simulink model "pulsar_channeliser"  (R2012b)
(part 2 of 105)

      mask prompts: vec_len "Vector length:"; arith_type "Output type:"; n_bits "Bit width (output):"; bin_pt "Binary point (output):"
      mask help: This simple vector accumulator is based on a shift register. It outputs its previous accumulated vector after a new_acc pulse is received.
      mask init:
      | simple_bram_vacc_init(gcb, ...
      |     'vec_len', vec_len, ...
      |     'arith_type', arith_type, ...
      |     'n_bits', n_bits, ...
      |     'bin_pt', bin_pt);
      mask TypeOptions arith_type: Signed | Unsigned
  simple_bram_vacc_q_odd : Subsystem  AncestorBlock=casper_library_accumulators/simple_bram_vacc  mask(simple_bram_vacc){vec_len=32, arith_type=Signed, n_bits=32, bin_pt=17}
      mask prompts: vec_len "Vector length:"; arith_type "Output type:"; n_bits "Bit width (output):"; bin_pt "Binary point (output):"
      mask help: This simple vector accumulator is based on a shift register. It outputs its previous accumulated vector after a new_acc pulse is received.
      mask init:
      | simple_bram_vacc_init(gcb, ...
      |     'vec_len', vec_len, ...
      |     'arith_type', arith_type, ...
      |     'n_bits', n_bits, ...
      |     'bin_pt', bin_pt);
      mask TypeOptions arith_type: Signed | Unsigned
  spead_pack_btm : Subsystem  Tag=casper:spead_pack  AncestorBlock=casper_library_communications/spead_pack  mask(pkt_pack_mask){max_pkt_len_bits=10, header_ids=0x1601, 0x1700, header_ind_ids=0x1800, spead_msw=64, spead_lsw=40, spead_version=4, bytes_per_word=8}
      mask prompts: max_pkt_len_bits "Max pkt length, 2^? 64-bit words"; header_ids "SPEAD direct address IDs (decimal)"; header_ind_ids "SPEAD indirect address IDs (decimal)"; spead_msw "SPEAD Flavour (MSw)"; spead_lsw "SPEAD Flavour (LSw)"; spead_version "SPEAD version"; bytes_per_word "Word size, in bytes"
      mask help:
      | This block generates SPEAD-compliant packets from a datastream.
      |
      | Packets are created with a fixed header followed by a number of 64-bit items.
      |
      | Requires a 64-bit data stream.
      |
      | The data_ready signal is one cycle BEFORE valid data! Does not have to be with a valid signal either.
      mask init:
      | if floor(log2(bytes_per_word)) ~= log2(bytes_per_word)
      |     error('Bytes per word should be a power of two.');
      | end
      | 
      | spead_pack_init(gcb)
  spead_pack_top : Subsystem  Tag=casper:spead_pack  AncestorBlock=casper_library_communications/spead_pack  mask(pkt_pack_mask){max_pkt_len_bits=10, header_ids=0x1601, 0x1700, header_ind_ids=0x1800, spead_msw=64, spead_lsw=40, spead_version=4, bytes_per_word=8}
      mask prompts: max_pkt_len_bits "Max pkt length, 2^? 64-bit words"; header_ids "SPEAD direct address IDs (decimal)"; header_ind_ids "SPEAD indirect address IDs (decimal)"; spead_msw "SPEAD Flavour (MSw)"; spead_lsw "SPEAD Flavour (LSw)"; spead_version "SPEAD version"; bytes_per_word "Word size, in bytes"
      mask help:
      | This block generates SPEAD-compliant packets from a datastream.
      |
      | Packets are created with a fixed header followed by a number of 64-bit items.
      |
      | Requires a 64-bit data stream.
      |
      | The data_ready signal is one cycle BEFORE valid data! Does not have to be with a valid signal either.
      mask init:
      | if floor(log2(bytes_per_word)) ~= log2(bytes_per_word)
      |     error('Bytes per word should be a power of two.');
      | end
      | 
      | spead_pack_init(gcb)
  status_reg_ctrl : Subsystem  Tag=xps:sw_reg  AncestorBlock=xps_library/software register  DataTypeOverride=Double  DataTypeOverrideAppliesTo=Fixed-point  MinMaxOverflowLogging=ForceOff  mask(swreg){mode=one value, io_dir=From Processor, io_delay=0, sample_period=1, names=of_reset, bitwidths=1, arith_types=2, bin_pts=0, sim_port=on, show_format=off}
      mask prompts: io_dir "I/O direction"; io_delay "I/O delay"; sample_period "Sample period"; names "Name:"; bitwidths "Bitwidth:"; arith_types "Type (ufix=0, fix=1, bool=2):"; bin_pts "Binary pt:"; sim_port "Provide sim input/output?"; show_format "Print format string?"
      mask init:
      | swreg_init(gcb)
      settings: AttributesFormatString=1input
      mask TypeOptions mode: one value | fields of equal size | fields of arbitrary size
      mask Callback mode: swreg_cb(gcb);
      mask TypeOptions io_dir: To Processor | From Processor
      mask Callback io_dir:
      | mask_enables = get_param(gcb, 'MaskEnables');
      | mask_names = get_param(gcb, 'MaskNames');
      | if strcmp(get_param(gcb, 'io_dir'), 'To Processor'),
      |     mask_enables{ismember(mask_names, 'sample_period')} = 'off';
      | else
      |     mask_enables{ismember(mask_names, 'sample_period')} = 'on';
      | end
      | set_param(gcb, 'MaskEnables', mask_enables);
      mask Callback bitwidths:
      | swreg_maskcheck(gcb);
      | % blk = gcb;
      | % mode = get_param(blk, 'mode');
      | % current_widths = eval(get_param(blk, 'bitwidths'));
      | % if (strcmp(mode, 'one value') || strcmp(mode, 'fields of equal size')) && (length(current_widths) > 1),
      | %     error('Only one width may be specified for this mode.');
      | % elseif strcmp(mode, 'fields of arbitrary size')
      | %     current_names = textscan(strtrim(strrep(strrep(get_param(blk, 'names'), ']', ''), '[', '')), '%s');
      | %     current_names = current_names{1};
      | %     numios = length(current_names);
      | %     if length(current_widths) ~= numios,
      | %         error('%d field names specified, but %d widths?', numios, length(current_widths));
      | %     end
      | % end
      | % total_width = 0;
      | % for ctr = 1 : length(current_widths),
      | %     total_width = total_width + current_widths(ctr);
      | % end
      | % if total_width > 32,
      | %     error('Total width must be 32 or less, set to %d.', total_width);
      | % end
      mask Callback arith_types:
      | [numios, ~, ~, ~, current_types] = swreg_maskcheck(gcb);
      | % blk = gcb;
      | % mode = get_param(blk, 'mode');
      | % current_types = eval(get_param(blk, 'arith_types'));
      | % numios = length(current_types);
      | % if (strcmp(mode, 'one value') || strcmp(mode, 'fields of equal size')) && (length(current_types) > 1),
      | %     error('Only one type may be specified for this mode.');
      | % elseif strcmp(mode, 'fields of arbitrary size')
      | %     current_names = textscan(strtrim(strrep(strrep(get_param(blk, 'names'), ']', ''), '[', '')), '%s');
      | %     current_names = current_names{1};
      | %     numios = length(current_names);
      | %     if length(current_types) ~= numios,
      | %         error('%d field names specified, but %d types?', numios, length(current_types));
      | %     end
      | % end
      | problem = 0;
      | for ctr = 1 : numios,
      |     t = current_types(ctr);
      |     if (t < 0) || (t > 2),
      |         problem = t;
      |         ctr = numios + 1;
      |     end
      | end
      | if problem ~= 0,
      |     error('Type cannot be %i, must be 0, 1 or 2.', problem);
      | end
      mask Callback bin_pts:
      | swreg_maskcheck(gcb);
      | % blk = gcb;
      | % mode = get_param(blk, 'mode');
      | % current_bins = eval(get_param(blk, 'bin_pts'));
      | % if (strcmp(mode, 'one value') || strcmp(mode, 'fields of equal size')) && (length(current_bins) > 1),
      | %     error('Only one binary pt may be specified for this mode.');
      | % elseif strcmp(mode, 'fields of arbitrary size')
      | %     current_names = textscan(strtrim(strrep(strrep(get_param(blk, 'names'), ']', ''), '[', '')), '%s');
      | %     current_names = current_names{1};
      | %     numios = length(current_names);
      | %     if length(current_bins) ~= numios,
      | %         error('%d field names specified, but %d binary pts?', numios, length(current_bins));
      | %     end
      | % end
  stokes_enable_true : xbsIndex_r4/Constant  const=1  gui_display_data_type=Boolean  arith_type=Boolean  n_bits=16  bin_pt=0  preci_type=Single  exp_width=8  frac_width=24  explicit_period=on  period=1  equ=P=C  opselect=C  inp2=PCIN>>17  opr=+  inp1=P  carry=CIN  dbl_ovrd=off  block_type=constant
  stokes_even : Subsystem
  stokes_odd : Subsystem
  stokes_snap : Subsystem  Tag=casper:bitsnap  AncestorBlock=casper_library_scopes/bitfield snapshot  mask(bitsnap){io_names=[lpower_even lpower_odd rpower_even rpower_odd], io_widths=[18 18 18 18], io_bps=[17 17 17 17], io_types=[1 1 1 1], show_format=on, snap_storage=bram, snap_dram_dimm=2, snap_dram_clock=250, snap_nsamples=10, snap_data_width=128, snap_offset=off, snap_circap=off, snap_value=off, snap_use_dsp48=on, snap_delay=0, extra_names=[c d], extra_widths=[30 2], extra_bps=[0 0], extra_types=[0 0]}
      mask prompts: io_names "Names [msb...lsb]"; io_widths "Bitwidths [msb...lsb]"; io_bps "Binary pts [msb...lsb]"; io_types "Data types [msb...lsb], ufix=0, fix=1, bool=2"; show_format "Print format string?"; snap_storage "Storage medium"; snap_dram_dimm "DRAM dimm"; snap_dram_clock "DRAM clock rate"; snap_nsamples "Number of Samples (2^?)"; snap_data_width "Data width"; snap_offset "Start delay support"; snap_circap "Circular capture support"; snap_value "Extra value capture support"; snap_use_dsp48 "Use DSP48s to implement counters"; snap_delay "Pre-snapshot delay"; extra_names "Names [msb...lsb]"; extra_widths "Widths [msb...lsb]"; extra_bps "Binary pts [msb...lsb]"; extra_types "Data types [msb...lsb], ufix=0, fix=1, bool=2"
      mask help:
      | A wrapped snapshot block. Allows specification of inputs to a snapblock word so the toolflow can automatically set up the scope.
      | See documentation for snapshot for explanation of parameters.
      mask init:
      | bitsnap_init(gcb);
      settings: AttributesFormatString=snap(4):f18.17,f18.17,f18.17,f18.17
      mask TypeOptions snap_storage: bram | dram
      mask Callback snap_storage: bitsnap_callback();
      mask TypeOptions snap_dram_dimm: 1 | 2 | 3 | 4
      mask TypeOptions snap_dram_clock: 200 | 250 | 266 | 300 | 333
      mask TypeOptions snap_data_width: 8 | 16 | 32 | 64 | 128
      mask Callback snap_value: bitsnap_callback();
  sub_frame_cnt : xbsIndex_r4/Counter  cnt_type=Free Running  cnt_to=Inf  operation=Up  start_count=0  cnt_by_val=1  arith_type=Unsigned  n_bits=8  bin_pt=0  load_pin=off  rst=on  en=on  explicit_period=on  period=1  dbl_ovrd=off  use_behavioral_HDL=off  implementation=Fabric  block_type=counter
      settings: block_version=11.4
  sync_ctrl : Subsystem  Tag=xps:sw_reg  AncestorBlock=xps_library/software register  DataTypeOverride=Double  DataTypeOverrideAppliesTo=Fixed-point  MinMaxOverflowLogging=ForceOff  mask(swreg){mode=one value, io_dir=From Processor, io_delay=0, sample_period=1, names=[arm self_pps sys_reset], bitwidths=[1 1 1], arith_types=[2 2 2], bin_pts=[0 0 0], sim_port=on, show_format=off}
      mask prompts: io_dir "I/O direction"; io_delay "I/O delay"; sample_period "Sample period"; names "Name:"; bitwidths "Bitwidth:"; arith_types "Type (ufix=0, fix=1, bool=2):"; bin_pts "Binary pt:"; sim_port "Provide sim input/output?"; show_format "Print format string?"
      mask init:
      | swreg_init(gcb)
      settings: AttributesFormatString=3 inputs
      mask TypeOptions mode: one value | fields of equal size | fields of arbitrary size
      mask Callback mode: swreg_cb(gcb);
      mask TypeOptions io_dir: To Processor | From Processor
      mask Callback io_dir:
      | mask_enables = get_param(gcb, 'MaskEnables');
      | mask_names = get_param(gcb, 'MaskNames');
      | if strcmp(get_param(gcb, 'io_dir'), 'To Processor'),
      |     mask_enables{ismember(mask_names, 'sample_period')} = 'off';
      | else
      |     mask_enables{ismember(mask_names, 'sample_period')} = 'on';
      | end
      | set_param(gcb, 'MaskEnables', mask_enables);
      mask Callback bitwidths:
      | swreg_maskcheck(gcb);
      | % blk = gcb;
      | % mode = get_param(blk, 'mode');
      | % current_widths = eval(get_param(blk, 'bitwidths'));
      | % if (strcmp(mode, 'one value') || strcmp(mode, 'fields of equal size')) && (length(current_widths) > 1),
      | %     error('Only one width may be specified for this mode.');
      | % elseif strcmp(mode, 'fields of arbitrary size')
      | %     current_names = textscan(strtrim(strrep(strrep(get_param(blk, 'names'), ']', ''), '[', '')), '%s');
      | %     current_names = current_names{1};
      | %     numios = length(current_names);
      | %     if length(current_widths) ~= numios,
      | %         error('%d field names specified, but %d widths?', numios, length(current_widths));
      | %     end
      | % end
      | % total_width = 0;
      | % for ctr = 1 : length(current_widths),
      | %     total_width = total_width + current_widths(ctr);
      | % end
      | % if total_width > 32,
      | %     error('Total width must be 32 or less, set to %d.', total_width);
      | % end
      mask Callback arith_types:
      | [numios, ~, ~, ~, current_types] = swreg_maskcheck(gcb);
      | % blk = gcb;
      | % mode = get_param(blk, 'mode');
      | % current_types = eval(get_param(blk, 'arith_types'));
      | % numios = length(current_types);
      | % if (strcmp(mode, 'one value') || strcmp(mode, 'fields of equal size')) && (length(current_types) > 1),
      | %     error('Only one type may be specified for this mode.');
      | % elseif strcmp(mode, 'fields of arbitrary size')
      | %     current_names = textscan(strtrim(strrep(strrep(get_param(blk, 'names'), ']', ''), '[', '')), '%s');
      | %     current_names = current_names{1};
      | %     numios = length(current_names);
      | %     if length(current_types) ~= numios,
      | %         error('%d field names specified, but %d types?', numios, length(current_types));
      | %     end
      | % end
      | problem = 0;
      | for ctr = 1 : numios,
      |     t = current_types(ctr);
      |     if (t < 0) || (t > 2),
      |         problem = t;
      |         ctr = numios + 1;
      |     end
      | end
      | if problem ~= 0,
      |     error('Type cannot be %i, must be 0, 1 or 2.', problem);
      | end
      mask Callback bin_pts:
      | swreg_maskcheck(gcb);
      | % blk = gcb;
      | % mode = get_param(blk, 'mode');
      | % current_bins = eval(get_param(blk, 'bin_pts'));
      | % if (strcmp(mode, 'one value') || strcmp(mode, 'fields of equal size')) && (length(current_bins) > 1),
      | %     error('Only one binary pt may be specified for this mode.');
      | % elseif strcmp(mode, 'fields of arbitrary size')
      | %     current_names = textscan(strtrim(strrep(strrep(get_param(blk, 'names'), ']', ''), '[', '')), '%s');
      | %     current_names = current_names{1};
      | %     numios = length(current_names);
      | %     if length(current_bins) ~= numios,
      | %         error('%d field names specified, but %d binary pts?', numios, length(current_bins));
      | %     end
      | % end
  sync_next_pps : Subsystem  Tag=xps:sw_reg  AncestorBlock=xps_library/software register  DataTypeOverride=Double  DataTypeOverrideAppliesTo=Fixed-point  MinMaxOverflowLogging=ForceOff  mask(swreg){mode=one value, io_dir=From Processor, io_delay=0, sample_period=1, names=reg, bitwidths=32, arith_types=0, bin_pts=[0], sim_port=on, show_format=off}
      mask prompts: io_dir "I/O direction"; io_delay "I/O delay"; sample_period "Sample period"; names "Name:"; bitwidths "Bitwidth:"; arith_types "Type (ufix=0, fix=1, bool=2):"; bin_pts "Binary pt:"; sim_port "Provide sim input/output?"; show_format "Print format string?"
      mask init:
      | swreg_init(gcb)
      settings: AttributesFormatString=1input
      mask TypeOptions mode: one value | fields of equal size | fields of arbitrary size
      mask Callback mode: swreg_cb(gcb);
      mask TypeOptions io_dir: To Processor | From Processor
      mask Callback io_dir:
      | mask_enables = get_param(gcb, 'MaskEnables');
      | mask_names = get_param(gcb, 'MaskNames');
      | if strcmp(get_param(gcb, 'io_dir'), 'To Processor'),
      |     mask_enables{ismember(mask_names, 'sample_period')} = 'off';
      | else
      |     mask_enables{ismember(mask_names, 'sample_period')} = 'on';
      | end
      | set_param(gcb, 'MaskEnables', mask_enables);
      mask Callback bitwidths:
      | swreg_maskcheck(gcb);
      | % blk = gcb;
      | % mode = get_param(blk, 'mode');
      | % current_widths = eval(get_param(blk, 'bitwidths'));
      | % if (strcmp(mode, 'one value') || strcmp(mode, 'fields of equal size')) && (length(current_widths) > 1),
      | %     error('Only one width may be specified for this mode.');
      | % elseif strcmp(mode, 'fields of arbitrary size')
      | %     current_names = textscan(strtrim(strrep(strrep(get_param(blk, 'names'), ']', ''), '[', '')), '%s');
      | %     current_names = current_names{1};
      | %     numios = length(current_names);
      | %     if length(current_widths) ~= numios,
      | %         error('%d field names specified, but %d widths?', numios, length(current_widths));
      | %     end
      | % end
      | % total_width = 0;
      | % for ctr = 1 : length(current_widths),
      | %     total_width = total_width + current_widths(ctr);
      | % end
      | % if total_width > 32,
      | %     error('Total width must be 32 or less, set to %d.', total_width);
      | % end
      mask Callback arith_types:
      | [numios, ~, ~, ~, current_types] = swreg_maskcheck(gcb);
      | % blk = gcb;
      | % mode = get_param(blk, 'mode');
      | % current_types = eval(get_param(blk, 'arith_types'));
      | % numios = length(current_types);
      | % if (strcmp(mode, 'one value') || strcmp(mode, 'fields of equal size')) && (length(current_types) > 1),
      | %     error('Only one type may be specified for this mode.');
      | % elseif strcmp(mode, 'fields of arbitrary size')
      | %     current_names = textscan(strtrim(strrep(strrep(get_param(blk, 'names'), ']', ''), '[', '')), '%s');
      | %     current_names = current_names{1};
      | %     numios = length(current_names);
      | %     if length(current_types) ~= numios,
      | %         error('%d field names specified, but %d types?', numios, length(current_types));
      | %     end
      | % end
      | problem = 0;
      | for ctr = 1 : numios,
      |     t = current_types(ctr);
      |     if (t < 0) || (t > 2),
      |         problem = t;
      |         ctr = numios + 1;
      |     end
      | end
      | if problem ~= 0,
      |     error('Type cannot be %i, must be 0, 1 or 2.', problem);
      | end
      mask Callback bin_pts:
      | swreg_maskcheck(gcb);
      | % blk = gcb;
      | % mode = get_param(blk, 'mode');
      | % current_bins = eval(get_param(blk, 'bin_pts'));
      | % if (strcmp(mode, 'one value') || strcmp(mode, 'fields of equal size')) && (length(current_bins) > 1),
      | %     error('Only one binary pt may be specified for this mode.');
      | % elseif strcmp(mode, 'fields of arbitrary size')
      | %     current_names = textscan(strtrim(strrep(strrep(get_param(blk, 'names'), ']', ''), '[', '')), '%s');
      | %     current_names = current_names{1};
      | %     numios = length(current_names);
      | %     if length(current_bins) ~= numios,
      | %         error('%d field names specified, but %d binary pts?', numios, length(current_bins));
      | %     end
      | % end
  tengbe0 : Subsystem  Tag=xps:tengbe_v2  AncestorBlock=xps_library/ten_Gbe_v2  mask(ten_GbE_v2){flavour=sfp+, slot=0, port_r1=0, port_r2_cx4=0, port_r2_sfpp=0, rx_dist_ram=on, large_frames=off, show_param=on, pre_emph_r2=1.07, pre_emph=3, post_emph_r2=0.18, rxeqmix_r2=7, swing_r2=940, swing=800, fab_en=on, fab_mac=hex2dec('123456780000'), fab_ip=10*(2^24) + 0*(2^16) + 0*(2^8) + 10*(2^0), fab_udp=60000, fab_gate=1, cpu_rx_en=on, cpu_tx_en=on, ttl=hex2dec('FF'), promisc_mode=off, debug_ctr_width=16, txctr=on, txerrctr=off, txerrctr_len=100, txofctr=on, txfullctr=off, txvldctr=on, txsnaplen=0 - no snap, rxctr=off, rxerrctr=off, rxerrctr_len=100, rxofctr=off, rxbadctr=off, rxvldctr=off, rxeofctr=off, rxsnaplen=0 - no snap}
      mask prompts: flavour "Mezzanine card flavour"; slot "Card slot"; port_r1 "Port"; port_r2_cx4 "Port"; port_r2_sfpp "Port"; rx_dist_ram "Shallow RX Fifo (Beware overruns!)"; large_frames "Enable Large TX Frames (8k+512)"; show_param "---------------------- Show Implementation Parameters -----------------------------------------------------------------------------------"; pre_emph_r2 "Pre-emphasis (dB)"; pre_emph "Pre-emphasis"; post_emph_r2 "Post-emphasis (dB)"; rxeqmix_r2 "Receive equalisation"; swing_r2 "Driver Swing Control (mVppd)"; swing "Differential swing"; fab_en "Enable fabric on startup"; fab_mac "Fabric MAC Address"; fab_ip "Fabric IP Address"; fab_udp "Fabric UDP Port"; fab_gate "Fabric Gateway"; cpu_rx_en "Enable CPU RX"; cpu_tx_en "Enable CPU TX"; promisc_mode "Promiscuous mode"; debug_ctr_width "Debug counter width"; txctr "TX - core_txctr"; txerrctr "TX packet length error - core_txerrctr"; txerrctr_len "-- expected TX packet length"; txofctr "TX overflow - core_txofctr"; txfullctr "TX full - core_txfullctr"; txvldctr "TX valid cycle - core_txvldctr"; txsnaplen "TX snapshot length"; rxctr "RX - core_rxctr"; rxerrctr "RX packet length error - core_rxerrctr"; rxerrctr_len "-- expected RX packet length"; rxofctr "RX overflow - core_rxofctr"; rxbadctr "RX bad - core_rxbadctr"; rxvldctr "RX valid cycle - core_rxvldctr"; rxeofctr "RX eof - core_rxeofctr"; rxsnaplen "RX snapshot length"
      mask help: This block sends and receives UDP frames (packets). It accepts a 64 bit wide data stream with user-determined frame breaks. The data stream is wrapped in a UDP frame for transmission. Incoming UDP packets are unwrapped and the data presented as a 64 bit wide stream.
      mask init:
      | temp = eval(get_param(gcb, 'debug_ctr_width'));
      | if temp <= 0,
      |     error('Debug counters cannot be ltoet zero.');
      | end
      | tengbe_v2_mask(gcb)
      mask TypeOptions flavour: sfp+ | cx4
      mask Callback flavour: tengbe_v2_callback
      mask TypeOptions slot: 0 | 1
      mask TypeOptions port_r1: 0 | 1 | 2 | 3
      mask TypeOptions port_r2_cx4: 0 | 1 | 2
      mask TypeOptions port_r2_sfpp: 0 | 1 | 2 | 3
      mask Callback show_param: tengbe_v2_callback
      mask TypeOptions pre_emph_r2: 0.15 | 0.3 | 0.45 | 0.61 | 0.74 | 0.91 | 1.07 | 1.25 | 1.36 | 1.55 | 1.74 | 1.94 | 2.11 | 2.32 | 2.54 | 2.77
      mask TypeOptions pre_emph: 0 | 1 | 2 | 3
      mask TypeOptions post_emph_r2: 0.18 | 0.19 | 0.2 | 0.39 | 0.63 | 0.82 | 1.07 | 1.32 | 1.6 | 1.65 | 1.94 | 2.21 | 2.52 | 2.76 | 3.08 | 3.41 | 3.77 | 3.97 | 4.36 | 4.73 | 5.16 | 5.47 | 5.93 | 6.38 | 6.89
      mask TypeOptions rxeqmix_r2: 0 | 1 | 2 | 3 | 4 | 5 | 6 | 7
      mask TypeOptions swing_r2: 110 | 210 | 310 | 400 | 480 | 570 | 660 | 740 | 810 | 880 | 940 | 990 | 1040 | 1080 | 1110 | 1130
      mask TypeOptions swing: 400 | 500 | 600 | 700 | 800
      mask Callback txerrctr:
      | blk = gcb;
      | mask_visibilities = get_param(blk, 'MaskVisibilities');
      | mask_names = get_param(blk, 'MaskNames');
      | if strcmp(get_param(blk, 'txerrctr'), 'on')
      |     mask_visibilities{ismember(mask_names, 'txerrctr_len')} = 'on';
      | else
      |     mask_visibilities{ismember(mask_names, 'txerrctr_len')} = 'off';
      | end
      | set_param(blk, 'MaskVisibilities', mask_visibilities);
      mask TypeOptions txsnaplen: 0 - no snap | 256 | 512 | 1024 | 2048 | 4096 | 8192 | 16384
      mask Callback rxerrctr:
      | blk = gcb;
      | mask_visibilities = get_param(blk, 'MaskVisibilities');
      | mask_names = get_param(blk, 'MaskNames');
      | if strcmp(get_param(blk, 'rxerrctr'), 'on')
      |     mask_visibilities{ismember(mask_names, 'rxerrctr_len')} = 'on';
      | else
      |     mask_visibilities{ismember(mask_names, 'rxerrctr_len')} = 'off';
      | end
      | set_param(blk, 'MaskVisibilities', mask_visibilities);
      mask TypeOptions rxsnaplen: 0 - no snap | 256 | 512 | 1024 | 2048 | 4096 | 8192 | 16384
  tengbe1 : Subsystem  Tag=xps:tengbe_v2  AncestorBlock=xps_library/ten_Gbe_v2  mask(ten_GbE_v2){flavour=sfp+, slot=0, port_r1=1, port_r2_cx4=0, port_r2_sfpp=0, rx_dist_ram=on, large_frames=off, show_param=on, pre_emph_r2=1.07, pre_emph=3, post_emph_r2=0.18, rxeqmix_r2=7, swing_r2=940, swing=800, fab_en=on, fab_mac=hex2dec('123456780001'), fab_ip=10*(2^24) + 0*(2^16) + 0*(2^8) + 20*(2^0), fab_udp=60000, fab_gate=1, cpu_rx_en=on, cpu_tx_en=on, ttl=hex2dec('FF'), promisc_mode=off, debug_ctr_width=16, txctr=on, txerrctr=off, txerrctr_len=100, txofctr=on, txfullctr=off, txvldctr=on, txsnaplen=0 - no snap, rxctr=off, rxerrctr=off, rxerrctr_len=100, rxofctr=off, rxbadctr=off, rxvldctr=off, rxeofctr=off, rxsnaplen=0 - no snap}
      mask prompts: flavour "Mezzanine card flavour"; slot "Card slot"; port_r1 "Port"; port_r2_cx4 "Port"; port_r2_sfpp "Port"; rx_dist_ram "Shallow RX Fifo (Beware overruns!)"; large_frames "Enable Large TX Frames (8k+512)"; show_param "---------------------- Show Implementation Parameters -----------------------------------------------------------------------------------"; pre_emph_r2 "Pre-emphasis (dB)"; pre_emph "Pre-emphasis"; post_emph_r2 "Post-emphasis (dB)"; rxeqmix_r2 "Receive equalisation"; swing_r2 "Driver Swing Control (mVppd)"; swing "Differential swing"; fab_en "Enable fabric on startup"; fab_mac "Fabric MAC Address"; fab_ip "Fabric IP Address"; fab_udp "Fabric UDP Port"; fab_gate "Fabric Gateway"; cpu_rx_en "Enable CPU RX"; cpu_tx_en "Enable CPU TX"; promisc_mode "Promiscuous mode"; debug_ctr_width "Debug counter width"; txctr "TX - core_txctr"; txerrctr "TX packet length error - core_txerrctr"; txerrctr_len "-- expected TX packet length"; txofctr "TX overflow - core_txofctr"; txfullctr "TX full - core_txfullctr"; txvldctr "TX valid cycle - core_txvldctr"; txsnaplen "TX snapshot length"; rxctr "RX - core_rxctr"; rxerrctr "RX packet length error - core_rxerrctr"; rxerrctr_len "-- expected RX packet length"; rxofctr "RX overflow - core_rxofctr"; rxbadctr "RX bad - core_rxbadctr"; rxvldctr "RX valid cycle - core_rxvldctr"; rxeofctr "RX eof - core_rxeofctr"; rxsnaplen "RX snapshot length"
      mask help: This block sends and receives UDP frames (packets). It accepts a 64 bit wide data stream with user-determined frame breaks. The data stream is wrapped in a UDP frame for transmission. Incoming UDP packets are unwrapped and the data presented as a 64 bit wide stream.
      mask init:
      | temp = eval(get_param(gcb, 'debug_ctr_width'));
      | if temp <= 0,
      |     error('Debug counters cannot be ltoet zero.');
      | end
      | tengbe_v2_mask(gcb)
      mask TypeOptions flavour: sfp+ | cx4
      mask Callback flavour: tengbe_v2_callback
      mask TypeOptions slot: 0 | 1
      mask TypeOptions port_r1: 0 | 1 | 2 | 3
      mask TypeOptions port_r2_cx4: 0 | 1 | 2
      mask TypeOptions port_r2_sfpp: 0 | 1 | 2 | 3
      mask Callback show_param: tengbe_v2_callback
      mask TypeOptions pre_emph_r2: 0.15 | 0.3 | 0.45 | 0.61 | 0.74 | 0.91 | 1.07 | 1.25 | 1.36 | 1.55 | 1.74 | 1.94 | 2.11 | 2.32 | 2.54 | 2.77
      mask TypeOptions pre_emph: 0 | 1 | 2 | 3
      mask TypeOptions post_emph_r2: 0.18 | 0.19 | 0.2 | 0.39 | 0.63 | 0.82 | 1.07 | 1.32 | 1.6 | 1.65 | 1.94 | 2.21 | 2.52 | 2.76 | 3.08 | 3.41 | 3.77 | 3.97 | 4.36 | 4.73 | 5.16 | 5.47 | 5.93 | 6.38 | 6.89
      mask TypeOptions rxeqmix_r2: 0 | 1 | 2 | 3 | 4 | 5 | 6 | 7
      mask TypeOptions swing_r2: 110 | 210 | 310 | 400 | 480 | 570 | 660 | 740 | 810 | 880 | 940 | 990 | 1040 | 1080 | 1110 | 1130
      mask TypeOptions swing: 400 | 500 | 600 | 700 | 800
      mask Callback txerrctr:
      | blk = gcb;
      | mask_visibilities = get_param(blk, 'MaskVisibilities');
      | mask_names = get_param(blk, 'MaskNames');
      | if strcmp(get_param(blk, 'txerrctr'), 'on')
      |     mask_visibilities{ismember(mask_names, 'txerrctr_len')} = 'on';
      | else
      |     mask_visibilities{ismember(mask_names, 'txerrctr_len')} = 'off';
      | end
      | set_param(blk, 'MaskVisibilities', mask_visibilities);
      mask TypeOptions txsnaplen: 0 - no snap | 256 | 512 | 1024 | 2048 | 4096 | 8192 | 16384
      mask Callback rxerrctr:
      | blk = gcb;
      | mask_visibilities = get_param(blk, 'MaskVisibilities');
      | mask_names = get_param(blk, 'MaskNames');
      | if strcmp(get_param(blk, 'rxerrctr'), 'on')
      |     mask_visibilities{ismember(mask_names, 'rxerrctr_len')} = 'on';
      | else
      |     mask_visibilities{ismember(mask_names, 'rxerrctr_len')} = 'off';
      | end
      | set_param(blk, 'MaskVisibilities', mask_visibilities);
      mask TypeOptions rxsnaplen: 0 - no snap | 256 | 512 | 1024 | 2048 | 4096 | 8192 | 16384
  tgbe0 : Subsystem  Tag=xps:tengbe_v2  AncestorBlock=xps_library/ten_Gbe_v2  mask(ten_GbE_v2){flavour=cx4, slot=1, port_r1=2, port_r2_cx4=0, port_r2_sfpp=0, rx_dist_ram=on, large_frames=off, show_param=on, pre_emph_r2=0.74, pre_emph=3, post_emph_r2=0.18, rxeqmix_r2=7, swing_r2=940, swing=800, fab_en=on, fab_mac=hex2dec('123456780000'), fab_ip=10*(2^24) + 0*(2^16) + 0*(2^8) + 2*(2^0), fab_udp=60001, fab_gate=1, cpu_rx_en=on, cpu_tx_en=on, ttl=hex2dec('FF'), promisc_mode=off, debug_ctr_width=16, txctr=on, txerrctr=off, txerrctr_len=4224, txofctr=on, txfullctr=off, txvldctr=on, txsnaplen=8192, rxctr=off, rxerrctr=off, rxerrctr_len=100, rxofctr=off, rxbadctr=off, rxvldctr=off, rxeofctr=off, rxsnaplen=0 - no snap}
      mask prompts: flavour "Mezzanine card flavour"; slot "Card slot"; port_r1 "Port"; port_r2_cx4 "Port"; port_r2_sfpp "Port"; rx_dist_ram "Shallow RX Fifo (Beware overruns!)"; large_frames "Enable Large TX Frames (8k+512)"; show_param "---------------------- Show Implementation Parameters -----------------------------------------------------------------------------------"; pre_emph_r2 "Pre-emphasis (dB)"; pre_emph "Pre-emphasis"; post_emph_r2 "Post-emphasis (dB)"; rxeqmix_r2 "Receive equalisation"; swing_r2 "Driver Swing Control (mVppd)"; swing "Differential swing"; fab_en "Enable fabric on startup"; fab_mac "Fabric MAC Address"; fab_ip "Fabric IP Address"; fab_udp "Fabric UDP Port"; fab_gate "Fabric Gateway"; cpu_rx_en "Enable CPU RX"; cpu_tx_en "Enable CPU TX"; promisc_mode "Promiscuous mode"; debug_ctr_width "Debug counter width"; txctr "TX - core_txctr"; txerrctr "TX packet length error - core_txerrctr"; txerrctr_len "-- expected TX packet length"; txofctr "TX overflow - core_txofctr"; txfullctr "TX full - core_txfullctr"; txvldctr "TX valid cycle - core_txvldctr"; txsnaplen "TX snapshot length"; rxctr "RX - core_rxctr"; rxerrctr "RX packet length error - core_rxerrctr"; rxerrctr_len "-- expected RX packet length"; rxofctr "RX overflow - core_rxofctr"; rxbadctr "RX bad - core_rxbadctr"; rxvldctr "RX valid cycle - core_rxvldctr"; rxeofctr "RX eof - core_rxeofctr"; rxsnaplen "RX snapshot length"
      mask help: This block sends and receives UDP frames (packets). It accepts a 64 bit wide data stream with user-determined frame breaks. The data stream is wrapped in a UDP frame for transmission. Incoming UDP packets are unwrapped and the data presented as a 64 bit wide stream.
      mask init:
      | temp = eval(get_param(gcb, 'debug_ctr_width'));
      | if temp <= 0,
      |     error('Debug counters cannot be ltoet zero.');
      | end
      | tengbe_v2_mask(gcb)
      mask TypeOptions flavour: sfp+ | cx4
      mask Callback flavour: tengbe_v2_callback
      mask TypeOptions slot: 0 | 1
      mask TypeOptions port_r1: 0 | 1 | 2 | 3
      mask TypeOptions port_r2_cx4: 0 | 1 | 2
      mask TypeOptions port_r2_sfpp: 0 | 1 | 2 | 3
      mask Callback show_param: tengbe_v2_callback
      mask TypeOptions pre_emph_r2: 0.15 | 0.3 | 0.45 | 0.61 | 0.74 | 0.91 | 1.07 | 1.25 | 1.36 | 1.55 | 1.74 | 1.94 | 2.11 | 2.32 | 2.54 | 2.77
      mask TypeOptions pre_emph: 0 | 1 | 2 | 3
      mask TypeOptions post_emph_r2: 0.18 | 0.19 | 0.2 | 0.39 | 0.63 | 0.82 | 1.07 | 1.32 | 1.6 | 1.65 | 1.94 | 2.21 | 2.52 | 2.76 | 3.08 | 3.41 | 3.77 | 3.97 | 4.36 | 4.73 | 5.16 | 5.47 | 5.93 | 6.38 | 6.89
      mask TypeOptions rxeqmix_r2: 0 | 1 | 2 | 3 | 4 | 5 | 6 | 7
      mask TypeOptions swing_r2: 110 | 210 | 310 | 400 | 480 | 570 | 660 | 740 | 810 | 880 | 940 | 990 | 1040 | 1080 | 1110 | 1130
      mask TypeOptions swing: 400 | 500 | 600 | 700 | 800
      mask Callback txerrctr:
      | blk = gcb;
      | mask_visibilities = get_param(blk, 'MaskVisibilities');
      | mask_names = get_param(blk, 'MaskNames');
      | if strcmp(get_param(blk, 'txerrctr'), 'on')
      |     mask_visibilities{ismember(mask_names, 'txerrctr_len')} = 'on';
      | else
      |     mask_visibilities{ismember(mask_names, 'txerrctr_len')} = 'off';
      | end
      | set_param(blk, 'MaskVisibilities', mask_visibilities);
      mask TypeOptions txsnaplen: 0 - no snap | 256 | 512 | 1024 | 2048 | 4096 | 8192 | 16384
      mask Callback rxerrctr:
      | blk = gcb;
      | mask_visibilities = get_param(blk, 'MaskVisibilities');
      | mask_names = get_param(blk, 'MaskNames');
      | if strcmp(get_param(blk, 'rxerrctr'), 'on')
      |     mask_visibilities{ismember(mask_names, 'rxerrctr_len')} = 'on';
      | else
      |     mask_visibilities{ismember(mask_names, 'rxerrctr_len')} = 'off';
      | end
      | set_param(blk, 'MaskVisibilities', mask_visibilities);
      mask TypeOptions rxsnaplen: 0 - no snap | 256 | 512 | 1024 | 2048 | 4096 | 8192 | 16384
  tgbe0_debug_reset : Subsystem  Tag=xps:sw_reg  AncestorBlock=xps_library/software register  mask(swreg){mode=one value, io_dir=From Processor, io_delay=0, sample_period=1, names=reg, bitwidths=32, arith_types=0, bin_pts=0, sim_port=on, show_format=off}
      mask prompts: io_dir "I/O direction"; io_delay "I/O delay"; sample_period "Sample period"; names "Name:"; bitwidths "Bitwidth:"; arith_types "Type (ufix=0, fix=1, bool=2):"; bin_pts "Binary pt:"; sim_port "Provide sim input/output?"; show_format "Print format string?"
      mask init:
      | swreg_init(gcb)
      settings: AttributesFormatString=1input
      mask TypeOptions mode: one value | fields of equal size | fields of arbitrary size
      mask Callback mode: swreg_cb(gcb);
      mask TypeOptions io_dir: To Processor | From Processor
      mask Callback io_dir:
      | mask_enables = get_param(gcb, 'MaskEnables');
      | mask_names = get_param(gcb, 'MaskNames');
      | if strcmp(get_param(gcb, 'io_dir'), 'To Processor'),
      |     mask_enables{ismember(mask_names, 'sample_period')} = 'off';
      | else
      |     mask_enables{ismember(mask_names, 'sample_period')} = 'on';
      | end
      | set_param(gcb, 'MaskEnables', mask_enables);
      mask Callback bitwidths: swreg_maskcheck(gcb);
      mask Callback arith_types: [numios, ~, ~, ~, current_types] = swreg_maskcheck(gcb);
      mask Callback bin_pts: swreg_maskcheck(gcb);
  tgbe0_dest_ip : Subsystem  Tag=xps:sw_reg  AncestorBlock=xps_library/software register  mask(swreg){mode=one value, io_dir=From Processor, io_delay=0, sample_period=1, names=reg, bitwidths=32, arith_types=0, bin_pts=0, sim_port=on, show_format=off}
      mask prompts: io_dir "I/O direction"; io_delay "I/O delay"; sample_period "Sample period"; names "Name:"; bitwidths "Bitwidth:"; arith_types "Type (ufix=0, fix=1, bool=2):"; bin_pts "Binary pt:"; sim_port "Provide sim input/output?"; show_format "Print format string?"
      mask init:
      | swreg_init(gcb)
      settings: AttributesFormatString=1input
      mask TypeOptions mode: one value | fields of equal size | fields of arbitrary size
      mask Callback mode: swreg_cb(gcb);
      mask TypeOptions io_dir: To Processor | From Processor
      mask Callback io_dir:
      | mask_enables = get_param(gcb, 'MaskEnables');
      | mask_names = get_param(gcb, 'MaskNames');
      | if strcmp(get_param(gcb, 'io_dir'), 'To Processor'),
      |     mask_enables{ismember(mask_names, 'sample_period')} = 'off';
      | else
      |     mask_enables{ismember(mask_names, 'sample_period')} = 'on';
      | end
      | set_param(gcb, 'MaskEnables', mask_enables);
      mask Callback bitwidths: swreg_maskcheck(gcb);
      mask Callback arith_types: [numios, ~, ~, ~, current_types] = swreg_maskcheck(gcb);
      mask Callback bin_pts: swreg_maskcheck(gcb);
  tgbe0_dest_port : Subsystem  Tag=xps:sw_reg  AncestorBlock=xps_library/software register  mask(swreg){mode=one value, io_dir=From Processor, io_delay=0, sample_period=1, names=reg, bitwidths=16, arith_types=0, bin_pts=0, sim_port=on, show_format=off}
      mask prompts: io_dir "I/O direction"; io_delay "I/O delay"; sample_period "Sample period"; names "Name:"; bitwidths "Bitwidth:"; arith_types "Type (ufix=0, fix=1, bool=2):"; bin_pts "Binary pt:"; sim_port "Provide sim input/output?"; show_format "Print format string?"
      mask init:
      | swreg_init(gcb)
      settings: AttributesFormatString=1input
      mask TypeOptions mode: one value | fields of equal size | fields of arbitrary size
      mask Callback mode: swreg_cb(gcb);
      mask TypeOptions io_dir: To Processor | From Processor
      mask Callback io_dir:
      | mask_enables = get_param(gcb, 'MaskEnables');
      | mask_names = get_param(gcb, 'MaskNames');
      | if strcmp(get_param(gcb, 'io_dir'), 'To Processor'),
      |     mask_enables{ismember(mask_names, 'sample_period')} = 'off';
      | else
      |     mask_enables{ismember(mask_names, 'sample_period')} = 'on';
      | end
      | set_param(gcb, 'MaskEnables', mask_enables);
      mask Callback bitwidths: swreg_maskcheck(gcb);
      mask Callback arith_types: [numios, ~, ~, ~, current_types] = swreg_maskcheck(gcb);
      mask Callback bin_pts: swreg_maskcheck(gcb);
  tgbe0_linkup : Subsystem  Tag=xps:sw_reg  AncestorBlock=xps_library/software register  mask(swreg){io_dir=To Processor, io_delay=0, sample_period=1, names=[top btm], bitwidths=[1 1], bin_pts=[0 0], arith_types=[2 2], sim_port=on, show_format=on}
      mask prompts: io_dir "I/O direction"; io_delay "I/O delay"; sample_period "Sample period"; names "Bitfield names [msb...lsb]"; bitwidths "Bitfield widths"; bin_pts "Bitfield binary pts"; arith_types "Bitfield types, ufix=0, fix=1, bool=2"; sim_port "Provide sim input/output?"; show_format "Print format string?"
      mask help: A 32-bit software-accessible register. Can be divided into bitfields of varying widths and types using the fields in the block mask.
      mask init:
      | swreg_init(gcb)
      settings: AttributesFormatString=2 outputs:b,b
      mask TypeOptions io_dir: To Processor | From Processor
      mask Callback io_dir:
      | mask_enables = get_param(gcb, 'MaskEnables');
      | mask_names = get_param(gcb, 'MaskNames');
      | if strcmp(get_param(gcb, 'io_dir'), 'To Processor'),
      |     mask_enables{ismember(mask_names, 'sample_period')} = 'off';
      | else
      |     mask_enables{ismember(mask_names, 'sample_period')} = 'on';
      | end
      | set_param(gcb, 'MaskEnables', mask_enables);
  tgbe0_linkup1 : Subsystem  Tag=xps:sw_reg  AncestorBlock=xps_library/software register  mask(swreg){mode=one value, io_dir=To Processor, io_delay=0, sample_period=1, names=reg, bitwidths=1, arith_types=2, bin_pts=0, sim_port=on, show_format=off}
      mask prompts: io_dir "I/O direction"; io_delay "I/O delay"; sample_period "Sample period"; names "Name:"; bitwidths "Bitwidth:"; arith_types "Type (ufix=0, fix=1, bool=2):"; bin_pts "Binary pt:"; sim_port "Provide sim input/output?"; show_format "Print format string?"
      mask init:
      | swreg_init(gcb)
      settings: AttributesFormatString=1output
      mask TypeOptions mode: one value | fields of equal size | fields of arbitrary size
      mask Callback mode: swreg_cb(gcb);
      mask TypeOptions io_dir: To Processor | From Processor
      mask Callback io_dir:
      | mask_enables = get_param(gcb, 'MaskEnables');
      | mask_names = get_param(gcb, 'MaskNames');
      | if strcmp(get_param(gcb, 'io_dir'), 'To Processor'),
      |     mask_enables{ismember(mask_names, 'sample_period')} = 'off';
      | else
      |     mask_enables{ismember(mask_names, 'sample_period')} = 'on';
      | end
      | set_param(gcb, 'MaskEnables', mask_enables);
      mask Callback bitwidths:
      | swreg_maskcheck(gcb);
      | % blk = gcb;
      | % mode = get_param(blk, 'mode');
      | % current_widths = eval(get_param(blk, 'bitwidths'));
      | % if (strcmp(mode, 'one value') || strcmp(mode, 'fields of equal size')) && (length(current_widths) > 1),
      | %     error('Only one width may be specified for this mode.');
      | % elseif strcmp(mode, 'fields of arbitrary size')
      | %     current_names = textscan(strtrim(strrep(strrep(get_param(blk, 'names'), ']', ''), '[', '')), '%s');
      | %     current_names = current_names{1};
      | %     numios = length(current_names);
      | %     if length(current_widths) ~= numios,
      | %         error('%d field names specified, but %d widths?', numios, length(current_widths));
      | %     end
      | % end
      | % total_width = 0;
      | % for ctr = 1 : length(current_widths),
      | %     total_width = total_width + current_widths(ctr);
      | % end
      | % if total_width > 32,
      | %     error('Total width must be 32 or less, set to %d.', total_width);
      | % end
      mask Callback arith_types:
      | [numios, ~, ~, ~, current_types] = swreg_maskcheck(gcb);
      | % blk = gcb;
      | % mode = get_param(blk, 'mode');
      | % current_types = eval(get_param(blk, 'arith_types'));
      | % numios = length(current_types);
      | % if (strcmp(mode, 'one value') || strcmp(mode, 'fields of equal size')) && (length(current_types) > 1),
      | %     error('Only one type may be specified for this mode.');
      | % elseif strcmp(mode, 'fields of arbitrary size')
      | %     current_names = textscan(strtrim(strrep(strrep(get_param(blk, 'names'), ']', ''), '[', '')), '%s');
      | %     current_names = current_names{1};
      | %     numios = length(current_names);
      | %     if length(current_types) ~= numios,
      | %         error('%d field names specified, but %d types?', numios, length(current_types));
      | %     end
      | % end
      | problem = 0;
      | for ctr = 1 : numios,
      |     t = current_types(ctr);
      |     if (t < 0) || (t > 2),
      |         problem = t;
      |         ctr = numios + 1;
      |     end
      | end
      | if problem ~= 0,
      |     error('Type cannot be %i, must be 0, 1 or 2.', problem);
      | end
      mask Callback bin_pts:
      | swreg_maskcheck(gcb);
      | % blk = gcb;
      | % mode = get_param(blk, 'mode');
      | % current_bins = eval(get_param(blk, 'bin_pts'));
      | % if (strcmp(mode, 'one value') || strcmp(mode, 'fields of equal size')) && (length(current_bins) > 1),
      | %     error('Only one binary pt may be specified for this mode.');
      | % elseif strcmp(mode, 'fields of arbitrary size')
      | %     current_names = textscan(strtrim(strrep(strrep(get_param(blk, 'names'), ']', ''), '[', '')), '%s');
      | %     current_names = current_names{1};
      | %     numios = length(current_names);
      | %     if length(current_bins) ~= numios,
      | %         error('%d field names specified, but %d binary pts?', numios, length(current_bins));
      | %     end
      | % end
  tgbe0_tx : Subsystem  Tag=xps:sw_reg  AncestorBlock=xps_library/software register  mask(swreg){mode=one value, io_dir=To Processor, io_delay=0, sample_period=1, names=reg, bitwidths=1, arith_types=2, bin_pts=0, sim_port=on, show_format=off}
      mask prompts: io_dir "I/O direction"; io_delay "I/O delay"; sample_period "Sample period"; names "Name:"; bitwidths "Bitwidth:"; arith_types "Type (ufix=0, fix=1, bool=2):"; bin_pts "Binary pt:"; sim_port "Provide sim input/output?"; show_format "Print format string?"
      mask init:
      | swreg_init(gcb)
      settings: AttributesFormatString=1output
      mask TypeOptions mode: one value | fields of equal size | fields of arbitrary size
      mask Callback mode: swreg_cb(gcb);
      mask TypeOptions io_dir: To Processor | From Processor
      mask Callback io_dir:
      | mask_enables = get_param(gcb, 'MaskEnables');
      | mask_names = get_param(gcb, 'MaskNames');
      | if strcmp(get_param(gcb, 'io_dir'), 'To Processor'),
      |     mask_enables{ismember(mask_names, 'sample_period')} = 'off';
      | else
      |     mask_enables{ismember(mask_names, 'sample_period')} = 'on';
      | end
      | set_param(gcb, 'MaskEnables', mask_enables);
      mask Callback bitwidths:
      | swreg_maskcheck(gcb);
      | % blk = gcb;
      | % mode = get_param(blk, 'mode');
      | % current_widths = eval(get_param(blk, 'bitwidths'));
      | % if (strcmp(mode, 'one value') || strcmp(mode, 'fields of equal size')) && (length(current_widths) > 1),
      | %     error('Only one width may be specified for this mode.');
      | % elseif strcmp(mode, 'fields of arbitrary size')
      | %     current_names = textscan(strtrim(strrep(strrep(get_param(blk, 'names'), ']', ''), '[', '')), '%s');
      | %     current_names = current_names{1};
      | %     numios = length(current_names);
      | %     if length(current_widths) ~= numios,
      | %         error('%d field names specified, but %d widths?', numios, length(current_widths));
      | %     end
      | % end
      | % total_width = 0;
      | % for ctr = 1 : length(current_widths),
      | %     total_width = total_width + current_widths(ctr);
      | % end
      | % if total_width > 32,
      | %     error('Total width must be 32 or less, set to %d.', total_width);
      | % end
      mask Callback arith_types:
      | [numios, ~, ~, ~, current_types] = swreg_maskcheck(gcb);
      | % blk = gcb;
      | % mode = get_param(blk, 'mode');
      | % current_types = eval(get_param(blk, 'arith_types'));
      | % numios = length(current_types);
      | % if (strcmp(mode, 'one value') || strcmp(mode, 'fields of equal size')) && (length(current_types) > 1),
      | %     error('Only one type may be specified for this mode.');
      | % elseif strcmp(mode, 'fields of arbitrary size')
      | %     current_names = textscan(strtrim(strrep(strrep(get_param(blk, 'names'), ']', ''), '[', '')), '%s');
      | %     current_names = current_names{1};
      | %     numios = length(current_names);
      | %     if length(current_types) ~= numios,
      | %         error('%d field names specified, but %d types?', numios, length(current_types));
      | %     end
      | % end
      | problem = 0;
      | for ctr = 1 : numios,
      |     t = current_types(ctr);
      |     if (t < 0) || (t > 2),
      |         problem = t;
      |         ctr = numios + 1;
      |     end
      | end
      | if problem ~= 0,
      |     error('Type cannot be %i, must be 0, 1 or 2.', problem);
      | end
      mask Callback bin_pts:
      | swreg_maskcheck(gcb);
      | % blk = gcb;
      | % mode = get_param(blk, 'mode');
      | % current_bins = eval(get_param(blk, 'bin_pts'));
      | % if (strcmp(mode, 'one value') || strcmp(mode, 'fields of equal size')) && (length(current_bins) > 1),
      | %     error('Only one binary pt may be specified for this mode.');
      | % elseif strcmp(mode, 'fields of arbitrary size')
      | %     current_names = textscan(strtrim(strrep(strrep(get_param(blk, 'names'), ']', ''), '[', '')), '%s');
      | %     current_names = current_names{1};
      | %     numios = length(current_names);
      | %     if length(current_bins) ~= numios,
      | %         error('%d field names specified, but %d binary pts?', numios, length(current_bins));
      | %     end
      | % end
  tgbe0_tx_full : Subsystem  Tag=xps:sw_reg  AncestorBlock=xps_library/software register  mask(swreg){mode=one value, io_dir=To Processor, io_delay=0, sample_period=1, names=reg, bitwidths=1, arith_types=2, bin_pts=0, sim_port=on, show_format=off}
      mask prompts: io_dir "I/O direction"; io_delay "I/O delay"; sample_period "Sample period"; names "Name:"; bitwidths "Bitwidth:"; arith_types "Type (ufix=0, fix=1, bool=2):"; bin_pts "Binary pt:"; sim_port "Provide sim input/output?"; show_format "Print format string?"
      mask init:
      | swreg_init(gcb)
      settings: AttributesFormatString=1output
      mask TypeOptions mode: one value | fields of equal size | fields of arbitrary size
      mask Callback mode: swreg_cb(gcb);
      mask TypeOptions io_dir: To Processor | From Processor
      mask Callback io_dir:
      | mask_enables = get_param(gcb, 'MaskEnables');
      | mask_names = get_param(gcb, 'MaskNames');
      | if strcmp(get_param(gcb, 'io_dir'), 'To Processor'),
      |     mask_enables{ismember(mask_names, 'sample_period')} = 'off';
      | else
      |     mask_enables{ismember(mask_names, 'sample_period')} = 'on';
      | end
      | set_param(gcb, 'MaskEnables', mask_enables);
      mask Callback bitwidths:
      | swreg_maskcheck(gcb);
      | % blk = gcb;
      | % mode = get_param(blk, 'mode');
      | % current_widths = eval(get_param(blk, 'bitwidths'));
      | % if (strcmp(mode, 'one value') || strcmp(mode, 'fields of equal size')) && (length(current_widths) > 1),
      | %     error('Only one width may be specified for this mode.');
      | % elseif strcmp(mode, 'fields of arbitrary size')
      | %     current_names = textscan(strtrim(strrep(strrep(get_param(blk, 'names'), ']', ''), '[', '')), '%s');
      | %     current_names = current_names{1};
      | %     numios = length(current_names);
      | %     if length(current_widths) ~= numios,
      | %         error('%d field names specified, but %d widths?', numios, length(current_widths));
      | %     end
      | % end
      | % total_width = 0;
      | % for ctr = 1 : length(current_widths),
      | %     total_width = total_width + current_widths(ctr);
      | % end
      | % if total_width > 32,
      | %     error('Total width must be 32 or less, set to %d.', total_width);
      | % end
      mask Callback arith_types:
      | [numios, ~, ~, ~, current_types] = swreg_maskcheck(gcb);
      | % blk = gcb;
      | % mode = get_param(blk, 'mode');
      | % current_types = eval(get_param(blk, 'arith_types'));
      | % numios = length(current_types);
      | % if (strcmp(mode, 'one value') || strcmp(mode, 'fields of equal size')) && (length(current_types) > 1),
      | %     error('Only one type may be specified for this mode.');
      | % elseif strcmp(mode, 'fields of arbitrary size')
      | %     current_names = textscan(strtrim(strrep(strrep(get_param(blk, 'names'), ']', ''), '[', '')), '%s');
      | %     current_names = current_names{1};
      | %     numios = length(current_names);
      | %     if length(current_types) ~= numios,
      | %         error('%d field names specified, but %d types?', numios, length(current_types));
      | %     end
      | % end
      | problem = 0;
      | for ctr = 1 : numios,
      |     t = current_types(ctr);
      |     if (t < 0) || (t > 2),
      |         problem = t;
      |         ctr = numios + 1;
      |     end
      | end
      | if problem ~= 0,
      |     error('Type cannot be %i, must be 0, 1 or 2.', problem);
      | end
      mask Callback bin_pts:
      | swreg_maskcheck(gcb);
      | % blk = gcb;
      | % mode = get_param(blk, 'mode');
      | % current_bins = eval(get_param(blk, 'bin_pts'));
      | % if (strcmp(mode, 'one value') || strcmp(mode, 'fields of equal size')) && (length(current_bins) > 1),
      | %     error('Only one binary pt may be specified for this mode.');
      | % elseif strcmp(mode, 'fields of arbitrary size')
      | %     current_names = textscan(strtrim(strrep(strrep(get_param(blk, 'names'), ']', ''), '[', '')), '%s');
      | %     current_names = current_names{1};
      | %     numios = length(current_names);
      | %     if length(current_bins) ~= numios,
      | %         error('%d field names specified, but %d binary pts?', numios, length(current_bins));
      | %     end
      | % end
  tgbe0_tx_of : Subsystem  Tag=xps:sw_reg  AncestorBlock=xps_library/software register  mask(swreg){mode=one value, io_dir=To Processor, io_delay=0, sample_period=1, names=reg, bitwidths=1, arith_types=2, bin_pts=0, sim_port=on, show_format=off}
      mask prompts: io_dir "I/O direction"; io_delay "I/O delay"; sample_period "Sample period"; names "Name:"; bitwidths "Bitwidth:"; arith_types "Type (ufix=0, fix=1, bool=2):"; bin_pts "Binary pt:"; sim_port "Provide sim input/output?"; show_format "Print format string?"
      mask init:
      | swreg_init(gcb)
      settings: AttributesFormatString=1output
      mask TypeOptions mode: one value | fields of equal size | fields of arbitrary size
      mask Callback mode: swreg_cb(gcb);
      mask TypeOptions io_dir: To Processor | From Processor
      mask Callback io_dir:
      | mask_enables = get_param(gcb, 'MaskEnables');
      | mask_names = get_param(gcb, 'MaskNames');
      | if strcmp(get_param(gcb, 'io_dir'), 'To Processor'),
      |     mask_enables{ismember(mask_names, 'sample_period')} = 'off';
      | else
      |     mask_enables{ismember(mask_names, 'sample_period')} = 'on';
      | end
      | set_param(gcb, 'MaskEnables', mask_enables);
      mask Callback bitwidths:
      | swreg_maskcheck(gcb);
      | % blk = gcb;
      | % mode = get_param(blk, 'mode');
      | % current_widths = eval(get_param(blk, 'bitwidths'));
      | % if (strcmp(mode, 'one value') || strcmp(mode, 'fields of equal size')) && (length(current_widths) > 1),
      | %     error('Only one width may be specified for this mode.');
      | % elseif strcmp(mode, 'fields of arbitrary size')
      | %     current_names = textscan(strtrim(strrep(strrep(get_param(blk, 'names'), ']', ''), '[', '')), '%s');
      | %     current_names = current_names{1};
      | %     numios = length(current_names);
      | %     if length(current_widths) ~= numios,
      | %         error('%d field names specified, but %d widths?', numios, length(current_widths));
      | %     end
      | % end
      | % total_width = 0;
      | % for ctr = 1 : length(current_widths),
      | %     total_width = total_width + current_widths(ctr);
      | % end
      | % if total_width > 32,
      | %     error('Total width must be 32 or less, set to %d.', total_width);
      | % end
      mask Callback arith_types:
      | [numios, ~, ~, ~, current_types] = swreg_maskcheck(gcb);
      | % blk = gcb;
      | % mode = get_param(blk, 'mode');
      | % current_types = eval(get_param(blk, 'arith_types'));
      | % numios = length(current_types);
      | % if (strcmp(mode, 'one value') || strcmp(mode, 'fields of equal size')) && (length(current_types) > 1),
      | %     error('Only one type may be specified for this mode.');
      | % elseif strcmp(mode, 'fields of arbitrary size')
      | %     current_names = textscan(strtrim(strrep(strrep(get_param(blk, 'names'), ']', ''), '[', '')), '%s');
      | %     current_names = current_names{1};
      | %     numios = length(current_names);
      | %     if length(current_types) ~= numios,
      | %         error('%d field names specified, but %d types?', numios, length(current_types));
      | %     end
      | % end
      | problem = 0;
      | for ctr = 1 : numios,
      |     t = current_types(ctr);
      |     if (t < 0) || (t > 2),
      |         problem = t;
      |         ctr = numios + 1;
      |     end
      | end
      | if problem ~= 0,
      |     error('Type cannot be %i, must be 0, 1 or 2.', problem);
      | end
      mask Callback bin_pts:
      | swreg_maskcheck(gcb);
      | % blk = gcb;
      | % mode = get_param(blk, 'mode');
      | % current_bins = eval(get_param(blk, 'bin_pts'));
      | % if (strcmp(mode, 'one value') || strcmp(mode, 'fields of equal size')) && (length(current_bins) > 1),
      | %     error('Only one binary pt may be specified for this mode.');
      | % elseif strcmp(mode, 'fields of arbitrary size')
      | %     current_names = textscan(strtrim(strrep(strrep(get_param(blk, 'names'), ']', ''), '[', '')), '%s');
      | %     current_names = current_names{1};
      | %     numios = length(current_names);
      | %     if length(current_bins) ~= numios,
      | %         error('%d field names specified, but %d binary pts?', numios, length(current_bins));
      | %     end
      | % end
  time_lsb : Subsystem  Tag=xps:sw_reg  AncestorBlock=xps_library/software register  DataTypeOverride=Double  DataTypeOverrideAppliesTo=Fixed-point  MinMaxOverflowLogging=ForceOff  mask(swreg){mode=one value, io_dir=From Processor, io_delay=0, sample_period=1, names=reg, bitwidths=32, arith_types=0, bin_pts=[0], sim_port=on, show_format=off}
      mask prompts: io_dir "I/O direction"; io_delay "I/O delay"; sample_period "Sample period"; names "Name:"; bitwidths "Bitwidth:"; arith_types "Type (ufix=0, fix=1, bool=2):"; bin_pts "Binary pt:"; sim_port "Provide sim input/output?"; show_format "Print format string?"
      mask init:
      | swreg_init(gcb)
      settings: AttributesFormatString=1input
      mask TypeOptions mode: one value | fields of equal size | fields of arbitrary size
      mask Callback mode: swreg_cb(gcb);
      mask TypeOptions io_dir: To Processor | From Processor
      mask Callback io_dir:
      | mask_enables = get_param(gcb, 'MaskEnables');
      | mask_names = get_param(gcb, 'MaskNames');
      | if strcmp(get_param(gcb, 'io_dir'), 'To Processor'),
      |     mask_enables{ismember(mask_names, 'sample_period')} = 'off';
      | else
      |     mask_enables{ismember(mask_names, 'sample_period')} = 'on';
      | end
      | set_param(gcb, 'MaskEnables', mask_enables);
      mask Callback bitwidths:
      | swreg_maskcheck(gcb);
      | % blk = gcb;
      | % mode = get_param(blk, 'mode');
      | % current_widths = eval(get_param(blk, 'bitwidths'));
      | % if (strcmp(mode, 'one value') || strcmp(mode, 'fields of equal size')) && (length(current_widths) > 1),
      | %     error('Only one width may be specified for this mode.');
      | % elseif strcmp(mode, 'fields of arbitrary size')
      | %     current_names = textscan(strtrim(strrep(strrep(get_param(blk, 'names'), ']', ''), '[', '')), '%s');
      | %     current_names = current_names{1};
      | %     numios = length(current_names);
      | %     if length(current_widths) ~= numios,
      | %         error('%d field names specified, but %d widths?', numios, length(current_widths));
      | %     end
      | % end
      | % total_width = 0;
      | % for ctr = 1 : length(current_widths),
      | %     total_width = total_width + current_widths(ctr);
      | % end
      | % if total_width > 32,
      | %     error('Total width must be 32 or less, set to %d.', total_width);
      | % end
      mask Callback arith_types:
      | [numios, ~, ~, ~, current_types] = swreg_maskcheck(gcb);
      | % blk = gcb;
      | % mode = get_param(blk, 'mode');
      | % current_types = eval(get_param(blk, 'arith_types'));
      | % numios = length(current_types);
      | % if (strcmp(mode, 'one value') || strcmp(mode, 'fields of equal size')) && (length(current_types) > 1),
      | %     error('Only one type may be specified for this mode.');
      | % elseif strcmp(mode, 'fields of arbitrary size')
      | %     current_names = textscan(strtrim(strrep(strrep(get_param(blk, 'names'), ']', ''), '[', '')), '%s');
      | %     current_names = current_names{1};
      | %     numios = length(current_names);
      | %     if length(current_types) ~= numios,
      | %         error('%d field names specified, but %d types?', numios, length(current_types));
      | %     end
      | % end
      | problem = 0;
      | for ctr = 1 : numios,
      |     t = current_types(ctr);
      |     if (t < 0) || (t > 2),
      |         problem = t;
      |         ctr = numios + 1;
      |     end
      | end
      | if problem ~= 0,
      |     error('Type cannot be %i, must be 0, 1 or 2.', problem);
      | end
      mask Callback bin_pts:
      | swreg_maskcheck(gcb);
      | % blk = gcb;
      | % mode = get_param(blk, 'mode');
      | % current_bins = eval(get_param(blk, 'bin_pts'));
      | % if (strcmp(mode, 'one value') || strcmp(mode, 'fields of equal size')) && (length(current_bins) > 1),
      | %     error('Only one binary pt may be specified for this mode.');
      | % elseif strcmp(mode, 'fields of arbitrary size')
      | %     current_names = textscan(strtrim(strrep(strrep(get_param(blk, 'names'), ']', ''), '[', '')), '%s');
      | %     current_names = current_names{1};
      | %     numios = length(current_names);
      | %     if length(current_bins) ~= numios,
      | %         error('%d field names specified, but %d binary pts?', numios, length(current_bins));
      | %     end
      | % end
  time_msb : Subsystem  Tag=xps:sw_reg  AncestorBlock=xps_library/software register  DataTypeOverride=Double  DataTypeOverrideAppliesTo=Fixed-point  MinMaxOverflowLogging=ForceOff  mask(swreg){mode=one value, io_dir=From Processor, io_delay=0, sample_period=1, names=reg, bitwidths=32, arith_types=0, bin_pts=[0], sim_port=on, show_format=off}
      mask prompts: io_dir "I/O direction"; io_delay "I/O delay"; sample_period "Sample period"; names "Name:"; bitwidths "Bitwidth:"; arith_types "Type (ufix=0, fix=1, bool=2):"; bin_pts "Binary pt:"; sim_port "Provide sim input/output?"; show_format "Print format string?"
      mask init:
      | swreg_init(gcb)
      settings: AttributesFormatString=1input
      mask TypeOptions mode: one value | fields of equal size | fields of arbitrary size
      mask Callback mode: swreg_cb(gcb);
      mask TypeOptions io_dir: To Processor | From Processor
      mask Callback io_dir:
      | mask_enables = get_param(gcb, 'MaskEnables');
      | mask_names = get_param(gcb, 'MaskNames');
      | if strcmp(get_param(gcb, 'io_dir'), 'To Processor'),
      |     mask_enables{ismember(mask_names, 'sample_period')} = 'off';
      | else
      |     mask_enables{ismember(mask_names, 'sample_period')} = 'on';
      | end
      | set_param(gcb, 'MaskEnables', mask_enables);
      mask Callback bitwidths:
      | swreg_maskcheck(gcb);
      | % blk = gcb;
      | % mode = get_param(blk, 'mode');
      | % current_widths = eval(get_param(blk, 'bitwidths'));
      | % if (strcmp(mode, 'one value') || strcmp(mode, 'fields of equal size')) && (length(current_widths) > 1),
      | %     error('Only one width may be specified for this mode.');
      | % elseif strcmp(mode, 'fields of arbitrary size')
      | %     current_names = textscan(strtrim(strrep(strrep(get_param(blk, 'names'), ']', ''), '[', '')), '%s');
      | %     current_names = current_names{1};
      | %     numios = length(current_names);
      | %     if length(current_widths) ~= numios,
      | %         error('%d field names specified, but %d widths?', numios, length(current_widths));
      | %     end
      | % end
      | % total_width = 0;
      | % for ctr = 1 : length(current_widths),
      | %     total_width = total_width + current_widths(ctr);
      | % end
      | % if total_width > 32,
      | %     error('Total width must be 32 or less, set to %d.', total_width);
      | % end
      mask Callback arith_types:
      | [numios, ~, ~, ~, current_types] = swreg_maskcheck(gcb);
      | % blk = gcb;
      | % mode = get_param(blk, 'mode');
      | % current_types = eval(get_param(blk, 'arith_types'));
      | % numios = length(current_types);
      | % if (strcmp(mode, 'one value') || strcmp(mode, 'fields of equal size')) && (length(current_types) > 1),
      | %     error('Only one type may be specified for this mode.');
      | % elseif strcmp(mode, 'fields of arbitrary size')
      | %     current_names = textscan(strtrim(strrep(strrep(get_param(blk, 'names'), ']', ''), '[', '')), '%s');
      | %     current_names = current_names{1};
      | %     numios = length(current_names);
      | %     if length(current_types) ~= numios,
      | %         error('%d field names specified, but %d types?', numios, length(current_types));
      | %     end
      | % end
      | problem = 0;
      | for ctr = 1 : numios,
      |     t = current_types(ctr);
      |     if (t < 0) || (t > 2),
      |         problem = t;
      |         ctr = numios + 1;
      |     end
      | end
      | if problem ~= 0,
      |     error('Type cannot be %i, must be 0, 1 or 2.', problem);
      | end
      mask Callback bin_pts:
      | swreg_maskcheck(gcb);
      | % blk = gcb;
      | % mode = get_param(blk, 'mode');
      | % current_bins = eval(get_param(blk, 'bin_pts'));
      | % if (strcmp(mode, 'one value') || strcmp(mode, 'fields of equal size')) && (length(current_bins) > 1),
      | %     error('Only one binary pt may be specified for this mode.');
      | % elseif strcmp(mode, 'fields of arbitrary size')
      | %     current_names = textscan(strtrim(strrep(strrep(get_param(blk, 'names'), ']', ''), '[', '')), '%s');
      | %     current_names = current_names{1};
      | %     numios = length(current_names);
      | %     if length(current_bins) ~= numios,
      | %         error('%d field names specified, but %d binary pts?', numios, length(current_bins));
      | %     end
      | % end
  timing : Subsystem  mask{reset_period=1, sync_gen_bits=28}
      mask prompts: reset_period "Master reset time (sync pulses)"; sync_gen_bits "Size of sync generator counter (bits)"
  window_size : xbsIndex_r4/Constant  const=1024/2  gui_display_data_type=Fixed-point  arith_type=Signed (2's comp)  n_bits=16  bin_pt=0  preci_type=Single  exp_width=8  frac_width=24  explicit_period=off  period=1  equ=P=C  opselect=C  inp2=PCIN>>17  opr=+  inp1=P  carry=CIN  dbl_ovrd=off  block_type=constant
  window_size1 : xbsIndex_r4/Constant  const=200  gui_display_data_type=Fixed-point  arith_type=Unsigned  n_bits=32  bin_pt=0  preci_type=Single  exp_width=8  frac_width=24  explicit_period=off  period=1  equ=P=C  opselect=C  inp2=PCIN>>17  opr=+  inp1=P  carry=CIN  dbl_ovrd=off  block_type=constant
  xsg_core_config : xps_library/XSG core config  Tag=xps:xsg  hw_sys=ROACH:sx95t  clk_src=adc0_clk  ROACH_clk_src=adc0_clk  ROACH2_clk_src=sys_clk  MKDIG_clk_src=sys_clk  clk_rate=200  sample_period=1  synthesis_tool=XST
  wires:
  Band-Limited White Noise/1 -> katadc/1(sim_data0), katadc/2(sim_data1)
  Pulse Generator/1 -> katadc/3(sim_sync)
  Constant/1 -> katadc/4(sim_data_valid)
  [sync] -> pfb_fir_real/1(sync)
  pfb_fir_real/9(pol2_out4) -> fft_wideband_real/10(in13)
  pfb_fir_real/8(pol2_out3) -> fft_wideband_real/9(in12)
  pfb_fir_real/7(pol2_out2) -> fft_wideband_real/8(in11)
  pfb_fir_real/6(pol2_out1) -> fft_wideband_real/7(in10)
  pfb_fir_real/5(pol1_out4) -> fft_wideband_real/6(in03)
  pfb_fir_real/4(pol1_out3) -> fft_wideband_real/5(in02)
  pfb_fir_real/3(pol1_out2) -> fft_wideband_real/4(in01)
  pfb_fir_real/2(pol1_out1) -> fft_wideband_real/3(in00)
  pfb_fir_real/1(sync_out) -> fft_wideband_real/1(sync)
  fft_wideband_real/1(sync_out) -> [fft_sync]
  sync_ctrl/2(in_self_pps) -> Delay10/1
  Constant10/1 -> Delay38/1
  Counter2/1 -> Delay37/1
  Relational/1 -> Delay42/1
  posedge1/1(out) -> Delay43/1
  katadc/5(or0) -> Delay5/1
  katadc/10(or1) -> Delay7/1
  fft_wideband_real/6(of) -> [fftof]
  requant0/4(of) -> [requant0of]
  requant1/4(of) -> [requant1of]
  [master_reset] -> buffer/6(reset)
  Constant15/1 -> spead_pack_top/4(hdr_heap_id)
  buffer/7(heap_size) -> Delay26/1
  [heap_size] -> Convert1/1
  Constant16/1 -> spead_pack_top/6(hdr_heap_offset), spead_pack_top/10(hdr7_0x1800)
  [band_select] -> Convert4/1
  Constant20/1 -> spead_pack_btm/4(hdr_heap_id)
  [heap_size] -> Convert/1
  Constant21/1 -> spead_pack_btm/10(hdr7_0x1800), spead_pack_btm/6(hdr_heap_offset)
  [band_select] -> Convert5/1
  spead_pack_top/3(eof) -> tengbe0/6(tx_end_of_frame)
  spead_pack_top/2(valid_out) -> tengbe0/3(tx_valid)
  spead_pack_top/1(data_out) -> tengbe0/2(tx_data)
  spead_pack_btm/3(eof) -> tengbe1/6(tx_end_of_frame)
  spead_pack_btm/2(valid_out) -> tengbe1/3(tx_valid)
  spead_pack_btm/1(data_out) -> tengbe1/2(tx_data)
  dest_port_top/1(in_reg) -> tengbe0/5(tx_dest_port)
  dest_ip_top/1(in_reg) -> tengbe0/4(tx_dest_ip)
  dest_port_btm/1(in_reg) -> tengbe1/5(tx_dest_port)
  dest_ip_btm/1(in_reg) -> tengbe1/4(tx_dest_ip)
  [master_reset] -> tengbe1/1(rst)
  Constant31/1 -> tengbe0/7(rx_ack), tengbe0/8(rx_overrun_ack), tengbe0/9(debug_rst)
  [master_reset] -> tengbe0/1(rst)
  Convert/1 -> spead_pack_btm/7(hdr_pkt_len_words), spead_pack_btm/5(hdr_heap_size)
  Convert1/1 -> spead_pack_top/5(hdr_heap_size), spead_pack_top/7(hdr_pkt_len_words)
  [fft_shift] -> fft_wideband_real/2(shift)
  [requant_tvg_en] -> requant0/5(tvg_en)
  [requant_tvg_en] -> requant1/5(tvg_en)
  [requant_gain] -> requant0/2(gain)
  [requant_gain] -> requant1/2(gain)
  band_select_validation/1(Out1) -> Delay45/1
  [band_select] -> band_split/2(band_select)
  [band_select] -> buffer/2(band_select)
  posedge2/1(out) -> [arm]
  [arm] -> band_select_validation/2(allow_modify)
  katadc/1(data0_0) -> bus_create/1(in1)
  katadc/2(data0_1) -> bus_create/2(in2)
  katadc/3(data0_2) -> bus_create/3(in3)
  katadc/4(data0_3) -> bus_create/4(in4)
  katadc/9(data1_3) -> bus_create1/4(in4)
  katadc/8(data1_2) -> bus_create1/3(in3)
  katadc/7(data1_1) -> bus_create1/2(in2)
  katadc/6(data1_0) -> bus_create1/1(in1)
  bus_create/1(bus_out) -> Delay4/1
  bus_create1/1(bus_out) -> Delay6/1
  bus_expand/1(msb_out4) -> pfb_fir_real/2(pol1_in1)
  bus_expand/2(out3) -> pfb_fir_real/3(pol1_in2)
  bus_expand/3(out2) -> pfb_fir_real/4(pol1_in3)
  bus_expand/4(lsb_out1) -> pfb_fir_real/5(pol1_in4)
  bus_expand1/1(msb_out4) -> pfb_fir_real/6(pol2_in1)
  bus_expand1/2(out3) -> pfb_fir_real/7(pol2_in2)
  bus_expand1/3(out2) -> pfb_fir_real/8(pol2_in3)
  bus_expand1/4(lsb_out1) -> pfb_fir_real/9(pol2_in4)
  fft_wideband_real/2(out00) -> bus_create2/1(in1)
  fft_wideband_real/3(out01) -> bus_create2/2(in2)
  fft_wideband_real/4(out10) -> bus_create3/1(in1)
  fft_wideband_real/5(out11) -> bus_create3/2(in2)
  bus_create2/1(bus_out) -> [fft_LCP]
  bus_create3/1(bus_out) -> [fft_RCP]
  [fft_LCP] -> bus_expand2/1(bus_in)
  bus_expand2/1(msb_out2) -> requant0/3(in_even)
  bus_expand2/2(lsb_out1) -> requant0/4(in_odd)
  [fft_RCP] -> bus_expand3/1(bus_in)
  bus_expand3/1(msb_out2) -> requant1/3(in_even)
  bus_expand3/2(lsb_out1) -> requant1/4(in_odd)
  requant1/2(out_even) -> bus_create5/1(in1)
  requant1/3(out_odd) -> bus_create5/2(in2)
  requant0/2(out_even) -> bus_create4/1(in1)
  requant0/3(out_odd) -> bus_create4/2(in2)
  bus_create4/1(bus_out) -> [requant_LCP]
  bus_create5/1(bus_out) -> [requant_RCP]
  bus_expand4/1(msb_out2) -> band_split/3(pol0even)
  bus_expand4/2(lsb_out1) -> band_split/4(pol0odd)
  [requant_LCP] -> bus_expand4/1(bus_in)
  [requant_RCP] -> bus_expand5/1(bus_in)
  bus_expand5/1(msb_out2) -> band_split/5(pol1even)
  bus_expand5/2(lsb_out1) -> band_split/6(pol1odd)
  band_split/2(top_dv) -> [band_top_dv]
  band_split/3(bottom_dv) -> [band_btm_dv]
  band_split/4(data) -> [band_data]
  [band_top_dv] -> buffer/3(dv_top)
  [band_btm_dv] -> buffer/4(dv_bottom)
  [band_data] -> buffer/5(data_in)
  [fft_sync] -> requant0/1(sync)
  requant0/1(sync_out) -> [requant_sync]
  [requant_sync] -> band_split/1(sync)
  band_split/1(sync_out) -> [band_sync]
  [band_sync] -> buffer/1(sync_in)
  [fft_sync] -> requant1/1(sync)
  sync_ctrl/3(in_sys_reset) -> Delay9/1
  [data_adc_LCP] -> bus_expand/1(bus_in)
  [data_adc_RCP] -> bus_expand1/1(bus_in)
  Convert5/1 -> spead_pack_btm/9(hdr6_0x1700_DIR)
  roach_led0/1 -> Terminator27/1
  roach_led1/1 -> Terminator31/1
  roach_led2/1 -> Terminator32/1
  roach_led3/1 -> Terminator33/1
  roach_led4/1 -> Terminator37/1
  roach_led5/1 -> Terminator34/1
  roach_led6/1 -> Terminator36/1
  roach_led7/1 -> Terminator35/1
  Delay64/1 -> roach_led7/1
  Delay47/1 -> roach_led6/1
  Delay65/1 -> roach_led5/1
  Delay67/1 -> roach_led4/1
  Delay39/1 -> roach_led2/1
  Delay44/1 -> roach_led3/1
  Delay66/1 -> roach_led1/1
  Delay152/1 -> roach_led0/1
  [timing_pps] -> keep_high_approx_100ms/1(In1)
  tengbe0/1(led_up) -> [top_eth_up]
  tengbe1/1(led_up) -> [btm_eth_up]
  [adc0or] -> latch/1(set)
  [adc1or] -> latch1/1(set)
  tengbe0/5(tx_overflow) -> [tx0of]
  tengbe1/5(tx_overflow) -> [tx1of]
  spead_pack_top/4(data_overflow) -> [sp0of]
  spead_pack_btm/4(data_overflow) -> [sp1of]
  [sp0of] -> latch5/1(set)
  [requant1of] -> latch4/1(set)
  [requant0of] -> latch3/1(set)
  [fftof] -> latch2/1(set)
  [sp1of] -> latch6/1(set)
  Logical2/1 -> [overflow_led]
  [overflow_led] -> Delay152/1
  [clk_bad] -> Delay66/1
  keep_high_approx_100ms/1(Out1) -> Delay64/1
  [top_eth_up] -> Delay47/1
  [btm_eth_up] -> Delay65/1
  [use_self_pps] -> Delay67/1
  Constant6/1 -> Delay44/1, Delay39/1
  Constant27/1 -> tengbe1/8(rx_overrun_ack), tengbe1/7(rx_ack), tengbe1/9(debug_rst)
  bus_expand9/1(msb_out2) -> Logical2/3
  bus_expand9/2(lsb_out1) -> Logical2/4
  katadc/11(sync0) -> Logical/1
  katadc/12(sync1) -> Logical/2
  katadc/13(sync2) -> Logical/3
  katadc/14(sync3) -> Logical/4
  Logical/1 -> edge_detect/1
  edge_detect/1 -> [adc_pps]
  timing/2(sync) -> [sync]
  Constant8/1 -> timing/3(sync_period)
  timing/1(armed) -> [armed], Logical1/2
  [sys_reset] -> Logical1/1
  Delay4/1 -> [adc_LCP]
  Delay5/1 -> [adc0or]
  Delay6/1 -> [adc_RCP]
  Delay7/1 -> [adc1or]
  [adc_pps] -> Mux12/2
  [self_pps] -> Mux12/3
  Mux12/1 -> timing/4(pps_in)
  Concat/1 -> timing/2(data_in)
  [adc_RCP] -> Concat/3
  [adc_LCP] -> Concat/2
  [adc_pps] -> Concat/1
  sync_ctrl/1(in_arm) -> Delay11/1
  [arm] -> timing/1(arm)
  timing/3(data_out) -> bus_expand10/1(bus_in)
  bus_expand10/3(lsb_out1) -> [data_adc_RCP]
  bus_expand10/2(out2) -> [data_adc_LCP]
  bus_expand10/1(msb_out3) -> [timing_pps]
  Counter5/1 -> Register19/1
  Register19/1 -> clk_frequency/1(reg_out), Relational3/1, Relational4/1
  clk_frequency/1(sim_reg_out) -> Terminator10/1
  pps_cnt/1(sim_reg_out) -> Terminator2/1
  [master_reset] -> Counter6/1
  [armed] -> Concat21/1
  Counter6/1 -> Concat21/2
  Concat21/1 -> pps_cnt/1(reg_out)
  Constant36/1 -> Relational3/2
  Relational3/1 -> Logical21/1
  Logical21/1 -> [clk_bad]
  Constant37/1 -> Relational4/2
  Relational4/1 -> Logical21/2
  Delay2/1 -> [requant_tvg_en]
  Delay8/1 -> [fft_shift]
  Delay9/1 -> [sys_reset]
  Delay11/1 -> posedge2/1(in)
  buffer/1(sync_out_top) -> Delay20/1
  [buffer_sync_top] -> spead_pack_top/1(data64_ready)
  buffer/2(dv_out_top) -> Delay21/1
  [buffer_dv_top] -> spead_pack_top/2(data64_valid)
  buffer/3(dout_top) -> Delay22/1
  [buffer_data_top] -> spead_pack_top/3(data64)
  buffer/4(sync_out_btm) -> Delay23/1
  [buffer_sync_btm] -> spead_pack_btm/1(data64_ready)
  buffer/5(dv_out_btm) -> Delay24/1
  [buffer_dv_btm] -> spead_pack_btm/2(data64_valid)
  buffer/6(dout_btm) -> Delay25/1
  [buffer_data_btm] -> spead_pack_btm/3(data64)
  [buffer_dv_top] -> frame_counter/2(dv)
  [band_select] -> frame_counter/3(band_select)
  [master_reset] -> frame_counter/1(reset)
  Convert4/1 -> spead_pack_top/9(hdr6_0x1700_DIR)
  frame_counter/1(frame_count) -> Delay13/1
  [frame_count] -> spead_pack_top/8(hdr5_0x1601_DIR)
  [frame_count] -> spead_pack_btm/8(hdr5_0x1601_DIR)
  Logical4/1 -> Register19/2, Counter6/2, Counter5/1
  [timing_pps] -> Logical4/1
  [self_pps] -> Logical4/2
  Delay12/1 -> frame_count/1(reg_out)
  [frame_count] -> Delay12/1
  latch/1(out) -> Logical2/1, overflows/1(out_adc0or)
  latch1/1(out) -> Logical2/2, overflows/2(out_adc1or)
  latch2/1(out) -> bus_expand9/1(bus_in), overflows/3(out_fftof)
  latch3/1(out) -> Logical2/5, overflows/4(out_rq0of)
  latch4/1(out) -> Logical2/6, overflows/5(out_rq1of)
  latch5/1(out) -> Logical2/7, overflows/6(out_sp0of)
  latch6/1(out) -> Logical2/8, overflows/7(out_sp1of)
  latch7/1(out) -> Logical2/9, overflows/8(out_tx0of)
  latch8/1(out) -> Logical2/10, overflows/9(out_tx1of)
  tengbe0/3(led_tx) -> [top_eth_tx]
  tengbe1/3(led_tx) -> [btm_eth_tx]
  tengbe0/4(tx_afull) -> [top_eth_afull]
  tengbe1/4(tx_afull) -> [btm_eth_afull]
  Constant13/1 -> sync_ctrl/2(sim_2)
  Step1/1 -> Sum/1
  Step2/1 -> Sum/2
  Sum/1 -> sync_ctrl/1(sim_1)
  overflows/1(sim_out) -> Terminator3/1
  frame_count/1(sim_reg_out) -> Terminator1/1
  Logical1/1 -> [master_reset]
  [use_self_pps] -> Mux12/1
  self_pps_validation/1(Out1) -> [use_self_pps]
  [arm] -> self_pps_validation/2(allow_modify)
  Delay10/1 -> self_pps_validation/1(In1), Counter2/1
  Constant23/1 -> sync_ctrl/3(sim_3)
  [btm_eth_up] -> tgbe0_linkup/2(out_btm)
  [top_eth_up] -> tgbe0_linkup/1(out_top)
  tgbe0_linkup/1(sim_out) -> Terminator4/1
  tengbe0/2(led_rx) -> Terminator5/1
  tengbe0/12(rx_overrun) -> Terminator13/1
  tengbe0/11(rx_bad_frame) -> Terminator12/1
  tengbe0/10(rx_end_of_frame) -> Terminator11/1
  tengbe0/9(rx_source_port) -> Terminator9/1
  tengbe0/8(rx_source_ip) -> Terminator8/1
  tengbe0/7(rx_valid) -> Terminator7/1
  tengbe0/6(rx_data) -> Terminator6/1
  tengbe1/12(rx_overrun) -> Terminator16/1
  tengbe1/11(rx_bad_frame) -> Terminator15/1
  tengbe1/10(rx_end_of_frame) -> Terminator14/1
  tengbe1/9(rx_source_port) -> Terminator21/1
  tengbe1/8(rx_source_ip) -> Terminator20/1
  tengbe1/7(rx_valid) -> Terminator19/1
  tengbe1/6(rx_data) -> Terminator18/1
  tengbe1/2(led_rx) -> Terminator17/1
  katadc/15(data_valid) -> Terminator22/1
  Constant5/1 -> dest_ip_top/1(sim_1)
  Constant7/1 -> dest_port_top/1(sim_1)
  Constant9/1 -> dest_ip_btm/1(sim_1)
  Constant11/1 -> dest_port_btm/1(sim_1)
  [tx1of] -> latch8/1(set)
  [tx0of] -> latch7/1(set)
  status_reg_ctrl/1(in_of_reset) -> latch4/2(reset), latch8/2(reset), latch7/2(reset), latch6/2(reset), latch5/2(reset), latch3/2(reset), latch2/2(reset), latch1/2(reset), latch/2(reset)
  Constant12/1 -> status_reg_ctrl/1(sim_1)
  Delay/1 -> [buffer_sync_top]
  Delay13/1 -> [frame_count]
  Delay14/1 -> [buffer_dv_top]
  Delay15/1 -> [buffer_data_top]
  Delay16/1 -> [buffer_sync_btm]
  Delay17/1 -> [buffer_dv_btm]
  Delay18/1 -> [buffer_data_btm]
  Delay19/1 -> [heap_size]
  Delay22/1 -> Delay15/1
  Delay21/1 -> Delay14/1
  Delay26/1 -> Delay19/1
  Delay23/1 -> Delay16/1
  Delay20/1 -> Delay/1
  Delay25/1 -> Delay18/1
  Delay24/1 -> Delay17/1
  sampling_frequency_mhz/1(sim_out) -> Terminator46/1
  Constant24/1 -> Delay228/1
  Delay228/1 -> sampling_frequency_mhz/1(out_reg)
  coarse_fft_size_nsamp/1(sim_out) -> Terminator49/1
  Constant25/1 -> Delay241/1
  Delay241/1 -> coarse_fft_size_nsamp/1(out_reg)
  fine_fft_size_nsamp/1(sim_out) -> Terminator50/1
  Constant26/1 -> Delay242/1
  Delay242/1 -> fine_fft_size_nsamp/1(out_reg)
  accum_samples_per_clk/1(sim_out) -> Terminator54/1
  Constant22/1 -> Delay232/1
  Delay232/1 -> accum_samples_per_clk/1(out_reg)
  Constant29/1 -> coarse_fft_shift_mask/1(sim_1)
  coarse_fft_shift_mask/1(in_reg) -> Delay8/1
  Delay27/1 -> [requant_gain]
  Constant30/1 -> requant_gain/1(sim_1)
  requant_gain/1(in_reg) -> Delay27/1
  Constant32/1 -> coarse_channel_select/1(sim_1)
  coarse_channel_select/1(in_reg) -> Delay28/1
  Delay28/1 -> band_select_validation/1(In1)
  requant_tvg_en/1(in_reg) -> Delay2/1
  Constant14/1 -> requant_tvg_en/1(sim_1)
  adc0_en/1(in_reg) -> Delay30/1
  Constant1/1 -> adc0_en/1(sim_1)
  Constant17/1 -> adc1_en/1(sim_1)
  adc1_en/1(in_reg) -> Delay29/1
  Constant3/1 -> adc0_atten/1(sim_1)
  Constant18/1 -> adc1_atten/1(sim_1)
  adc1_atten/1(in_reg) -> Delay1/1
  adc0_atten/1(in_reg) -> Delay3/1
  Delay1/1 -> katadc/8(atten1)
  Delay3/1 -> katadc/6(atten0)
  Delay29/1 -> katadc/7(en1)
  Delay30/1 -> katadc/5(en0)
  noise_diode_en/1(sim_out) -> Terminator23/1
  Constant2/1 -> Delay31/1
  Delay31/1 -> noise_diode_en/1(out_reg)
  noise_diode_duty_cycle_en/1(sim_out) -> Terminator24/1
  Constant4/1 -> Delay32/1
  Delay32/1 -> noise_diode_duty_cycle_en/1(out_reg)
  noise_diode_on_length/1(sim_out) -> Terminator25/1
  Constant19/1 -> Delay33/1
  Delay33/1 -> noise_diode_on_length/1(out_reg)
  noise_diode_off_length/1(sim_out) -> Terminator26/1
  Constant28/1 -> Delay34/1
  Delay34/1 -> noise_diode_off_length/1(out_reg)
  c_to_ri/1 -> Delay95/1
  c_to_ri/2 -> Delay96/1
  c_to_ri1/1 -> Delay97/1
  c_to_ri1/2 -> Delay98/1
  c_to_ri2/1 -> Delay99/1
  c_to_ri2/2 -> Delay100/1
  c_to_ri3/1 -> Delay101/1
  c_to_ri3/2 -> Delay102/1
  [fft_sync] -> Delay103/1
  bus_expand6/1(msb_out2) -> c_to_ri/1
  bus_expand6/2(lsb_out1) -> c_to_ri2/1
  bus_expand7/1(msb_out2) -> c_to_ri1/1
  bus_expand7/2(lsb_out1) -> c_to_ri3/1
  Delay95/1 -> stokes_even/2(left_real)
  Delay96/1 -> stokes_even/3(left_imag)
  Delay97/1 -> stokes_even/4(right_real)
  Delay98/1 -> stokes_even/5(right_imag)
  Delay100/1 -> stokes_odd/3(left_imag)
  Delay101/1 -> stokes_odd/4(right_real)
  Delay102/1 -> stokes_odd/5(right_imag)
  stokes_even/1(sync_out) -> stokes_snap/6(trig), [stokes_sync_out]
  stokes_odd/1(sync_out) -> Terminator41/1
  Delay99/1 -> stokes_odd/2(left_real)
  Delay103/1 -> stokes_odd/1(sync_in), stokes_even/1(sync_in)
  [fft_LCP] -> bus_expand6/1(bus_in)
  [fft_RCP] -> bus_expand7/1(bus_in)
  simple_bram_vacc_i_even/2(valid) -> Delay83/1
  simple_bram_vacc_q_even/2(valid) -> Delay106/1
  Logical5/1 -> Logical7/1
  simple_bram_vacc_i_even/1(dout) -> Delay59/1
  simple_bram_vacc_q_even/1(dout) -> Delay105/1
  simple_bram_vacc_i_odd/2(valid) -> Delay133/1
  simple_bram_vacc_q_odd/2(valid) -> Delay135/1
  Logical6/1 -> Logical7/2
  simple_bram_vacc_i_odd/1(dout) -> Delay132/1
  simple_bram_vacc_q_odd/1(dout) -> Delay134/1
  data_bus/1(bus_out) -> Delay54/1
  Delay36/1 -> simple_bram_vacc_q_even/1(new_acc)
  Delay40/1 -> simple_bram_vacc_i_odd/1(new_acc)
  Delay41/1 -> simple_bram_vacc_q_odd/1(new_acc)
  Delay48/1 -> simple_bram_vacc_q_odd/2(din)
  Delay49/1 -> simple_bram_vacc_i_odd/2(din)
  Delay52/1 -> simple_bram_vacc_q_even/2(din)
  Delay35/1 -> simple_bram_vacc_i_even/1(new_acc)
  Delay54/1 -> packetizer/2(din)
  Logical7/1 -> [packetiser_din_v], Delay55/1
  packetizer/4(buffer_overflow) -> [packetiser_of]
  Delay55/1 -> packetizer/1(din_valid)
  packetizer/2(data_sout) -> Delay50/1, [packetiser_dout]
  packetizer/1(data_addr) -> [packetiser_addr]
  [acc_trig] -> Delay35/1
  [acc_trig] -> Delay36/1
  [acc_trig] -> Delay40/1
  [acc_trig] -> Delay41/1
  Delay105/1 -> Delay58/1, data_bus/4(in4), data_bus/2(in2)
  Delay106/1 -> Logical5/2
  Delay132/1 -> Delay69/1, data_bus/7(in7), data_bus/5(in5)
  Delay133/1 -> Logical6/1
  Delay134/1 -> Delay57/1, data_bus/8(in8), data_bus/6(in6)
  Delay135/1 -> Logical6/2
  packetizer/5(perc_full) -> [packetiser_perc_full]
  Delay56/1 -> packetizer/3(reset)
  [eth_reset] -> Delay56/1
  packetizer/6(done) -> [packetiser_done]
  Delay160/1 -> Delay53/1
  Delay161/1 -> Delay52/1
  Delay164/1 -> Delay49/1
  Delay165/1 -> Delay48/1
  Delay53/1 -> simple_bram_vacc_i_even/2(din)
  Delay207/1 -> Delay160/1
  Delay209/1 -> Delay161/1
  Delay221/1 -> Delay164/1
  Delay223/1 -> Delay165/1
  stokes_odd/3(r_power) -> stokes_snap/4(in_rpower_odd), Delay222/1
  Delay222/1 -> Delay223/1
  stokes_even/3(r_power) -> Delay208/1, stokes_snap/3(in_rpower_even)
  Delay208/1 -> Delay209/1
  stokes_even/2(l_power) -> stokes_snap/1(in_lpower_even), Delay150/1
  Delay150/1 -> Delay207/1
  stokes_odd/2(l_power) -> stokes_snap/2(in_lpower_odd), Delay220/1
  Delay220/1 -> Delay221/1
  [packetiser_dout_v] -> Delay113/1
  [packetiser_dout] -> Delay112/1
  Delay112/1 -> FIFO/1
  Delay113/1 -> FIFO/2
  Delay114/1 -> FIFO/4
  [eth_reset] -> Delay114/1
  [eth_data_tx_valid] -> FIFO/3
  FIFO/2 -> [queue_empty]
  FIFO/4 -> [queue_full]
  FIFO/1 -> [queue_dout]
  FIFO/3 -> [queue_perc_full]
  Signal Builder/1(Signal 1) -> eth_reset/1(sim_1)
  eth_reset/1(in_reg) -> Slice/1
  [packetiser_din_v] -> posedge11/1(in)
  Logical9/1 -> Counter12/1
  posedge12/1(out) -> Counter12/2
  Counter12/1 -> Slice6/1
  Slice6/1 -> Logical10/1
  Logical10/1 -> Delay177/1
  Inverter3/1 -> Logical9/2
  Delay68/1 -> posedge12/1(in), Logical10/2, Inverter3/1
  Logical15/1 -> Delay68/1
  Slice/1 -> Logical15/1
  [stokes_sync_out] -> Delay60/1
  Delay60/1 -> Logical15/2
  posedge11/1(out) -> Logical9/1
  Delay177/1 -> [eth_reset]
  magic_no/1 -> Concat4/1
  Concat6/1 -> Concat4/5
  [eth_reset] -> Delay144/1
  sub_frame_cnt/1 -> Concat4/3, [hdr_subframe_cnt], Relational6/1
  Logical8/1 -> sub_frame_cnt/1
  Delay144/1 -> Logical8/2
  [eth_eof] -> sub_frame_cnt/2
  Concat4/1 -> [hdr_dout]
  Relational6/1 -> Logical8/1
  [eth_packets_per_accum_window] -> Delay170/1
  Delay170/1 -> Concat4/4
  stokes_enable_true/1 -> Delay245/1
  another3/1 -> Concat6/1
  [timestamp] -> Reinterpret9/1
  Reinterpret9/1 -> Concat4/2
  another1/1 -> AddSub2/2
  [eth_packets_per_accum_window] -> Delay206/1
  AddSub2/1 -> Delay200/1
  Delay200/1 -> Relational6/2
  Delay206/1 -> AddSub2/1
  Delay245/1 -> Concat6/3
  another2/1 -> Concat6/2
  err_clear_sim4/1 -> tgbe0_dest_port/1(sim_1)
  tgbe0_dest_port/1(in_reg) -> Delay80/1
  err_clear_sim3/1 -> tgbe0_dest_ip/1(sim_1)
  tgbe0_dest_ip/1(in_reg) -> Delay79/1
  Constant33/1 -> tgbe0/8(rx_overrun_ack), tgbe0/7(rx_ack)
  tgbe0/6(rx_data) -> Terminator52/1
  tgbe0/7(rx_valid) -> Terminator53/1
  tgbe0/8(rx_source_ip) -> Terminator55/1
  tgbe0/9(rx_source_port) -> Terminator56/1
  tgbe0/1(led_up) -> Delay77/1, [eth_up]
  tgbe0/2(led_rx) -> Terminator48/1
  tgbe0/3(led_tx) -> Delay76/1
  Delay61/1 -> tgbe0_tx_of/1(out_reg)
  Delay63/1 -> tgbe0_tx_full/1(out_reg)
  Delay76/1 -> tgbe0_tx/1(out_reg)
  Delay77/1 -> tgbe0_linkup1/1(out_reg)
  Delay78/1 -> tgbe0/1(rst)
  Delay79/1 -> tgbe0/4(tx_dest_ip)
  Delay80/1 -> tgbe0/5(tx_dest_port)
  Mux/1 -> tgbe0/2(tx_data), [eth_tx_data]
  Logical20/1 -> Delay81/1
  [eth_reset] -> posedge13/1(in)
  tgbe0_linkup1/1(sim_out) -> Terminator47/1
  tgbe0_tx/1(sim_out) -> Terminator51/1
  tgbe0_tx_full/1(sim_out) -> Terminator44/1
  tgbe0_tx_of/1(sim_out) -> Terminator45/1
  posedge13/1(out) -> Delay78/1
  [eth_eof] -> Delay94/1
  tgbe0/4(tx_afull) -> Delay63/1
  Delay94/1 -> tgbe0/6(tx_end_of_frame)
  Delay141/1 -> Mux/2
  [hdr_dout] -> Slice9/1, Slice10/1
  Delay140/1 -> Mux/3
  Slice9/1 -> Delay141/1
  Slice10/1 -> Delay140/1
  [queue_dout] -> Delay62/1
  Concat5/1 -> Delay142/1, [eth_mux_select]
  [eth_hdr_tx_valid] -> Inverter4/1, Logical22/1
  Delay142/1 -> Mux/1
  Inverter4/1 -> Concat5/1
  [hdr_length_cnt] -> Slice11/1
  Logical22/1 -> Concat5/2
  Slice11/1 -> Logical22/2
  [eth_hdr_tx_valid] -> Logical20/2
  Delay81/1 -> tgbe0/3(tx_valid)
  [eth_data_tx_valid] -> Logical20/1
  Delay62/1 -> Mux/4
  tgbe0/5(tx_overflow) -> Delay61/1, [eth_tx_of]
  err_clear_sim1/1 -> tgbe0_debug_reset/1(sim_1)
  tgbe0_debug_reset/1(in_reg) -> Delay82/1
  Delay82/1 -> Slice7/1
  Slice7/1 -> tgbe0/9(debug_rst)
  tgbe0/10(rx_end_of_frame) -> Terminator59/1
  tgbe0/11(rx_bad_frame) -> Terminator57/1
  tgbe0/12(rx_overrun) -> Terminator58/1
  Counter3/1 -> Delay87/1, Delay91/1
  eth_eof_cnt/1(sim_out) -> Terminator60/1
  Delay87/1 -> eth_eof_cnt/1(out_reg)
  Delay89/1 -> Counter3/2
  [eth_reset] -> Delay90/1
  Delay90/1 -> Counter3/1
  [eth_eof] -> Delay89/1
  Delay91/1 -> Slice12/1
  Slice12/1 -> [eth_eof_led]
  accumlation_count1/1 -> digital_gain/1(sim_1)
  digital_gain/1(in_reg) -> Delay92/1
  Delay92/1 -> stokes_even/6(digital_gain), stokes_odd/6(digital_gain)
  accumulation_length/1(in_reg) -> Delay108/1
  accumlation_count/1 -> accumulation_length/1(sim_1)
  Relational1/1 -> Logical12/1, Logical13/2
  Counter4/1 -> Relational2/1, [clk_cnt]
  window_size/1 -> Relational2/2
  Relational2/1 -> Logical11/1, posedge3/1(in)
  posedge3/1(out) -> Delay147/1
  [stokes_sync_out] -> Logical11/2, Logical12/2, Delay93/1
  Logical11/1 -> Counter4/1
  Logical12/1 -> Counter7/1
  Logical13/1 -> posedge/1(in)
  Delay93/1 -> Logical13/1
  accumulation_cnt/1(sim_out) -> Terminator61/1
  Delay107/1 -> accumulation_cnt/1(out_reg), Slice1/1
  Delay108/1 -> Relational1/2
  Counter7/1 -> Delay107/1, Relational1/1
  acc_trig_cnt/1(sim_out) -> Terminator62/1
  Counter10/1 -> acc_trig_cnt/1(out_reg)
  posedge10/1(out) -> Counter10/1
  [acc_trig] -> posedge10/1(in)
  posedge/1(out) -> Delay151/1
  Slice1/1 -> [acc_trig_led]
  Delay147/1 -> Counter7/2
  Delay151/1 -> [acc_trig]
  posedge4/1(out) -> [eth_eof], Logical25/1
  Counter11/1 -> Relational5/1, [packet_length_cnt]
  Logical25/1 -> Counter11/1
  [queue_empty] -> Inverter6/1
  [eth_reset] -> Logical25/2
  Counter13/1 -> Relational7/1, [interpacket_length_cnt]
  Logical14/1 -> Counter13/1
  Delay116/1 -> Slice16/1
  Relational7/1 -> posedge14/1(in)
  [eth_reset] -> Logical14/2
  eth_interframe_length_/1 -> eth_interpacket_length/1(sim_1)
  eth_interpacket_length/1(in_reg) -> Delay116/1
  Logical16/1 -> [eth_data_tx_valid], Counter11/2
  Counter14/1 -> Slice13/1
  [eth_eof] -> Logical17/1
  Logical17/1 -> Counter14/2
  [hdr_send_end] -> Logical17/2
  [eth_eof] -> Logical18/1
  Logical18/1 -> Counter15/2
  [interpacket_end] -> Logical18/2
  Relational5/1 -> posedge4/1(in)
  [eth_reset] -> Counter14/1
  posedge14/1(out) -> [interpacket_end], Logical14/1
  [eth_reset] -> Counter15/1
  Counter15/1 -> Slice14/1
  Slice13/1 -> Logical16/2
  Slice14/1 -> Counter13/2, [interpacket_valid]
  Counter16/1 -> Relational8/1, [hdr_length_cnt]
  Logical23/1 -> Counter16/1
  hdr_size/1 -> Relational8/2
  Relational8/1 -> posedge8/1(in)
  [eth_reset] -> Logical23/2
  [interpacket_end] -> Logical24/1
  Logical24/1 -> Counter17/2
  [hdr_send_end] -> Logical24/2
  posedge8/1(out) -> [hdr_send_end], Logical23/1
  [eth_reset] -> Counter17/1
  Counter17/1 -> Slice8/1
  Slice8/1 -> Counter16/2, Logical19/1
  [eth_reset] -> Inverter5/1
  Inverter5/1 -> Logical19/2
  Logical19/1 -> [eth_hdr_tx_valid]
  Inverter6/1 -> Logical16/1
  Delay110/1 -> Slice17/1
  eth_interframe_length_1/1 -> eth_packets_per_accum_window/1(sim_1)
  eth_packets_per_accum_window/1(in_reg) -> Delay110/1
  "1 "/1 -> AddSub/2
  Slice16/1 -> Relational7/2
  Slice17/1 -> [eth_packets_per_accum_window]
  Shift/1 -> AddSub/1
  Delay171/1 -> Slice19/1
  eth_interframe_length_2/1 -> eth_data_size_per_packet/1(sim_1)
  eth_data_size_per_packet/1(in_reg) -> Delay171/1
  Slice19/1 -> [eth_data_size_per_packet]
  eth_cycles_per_packet/1(sim_out) -> Terminator63/1
  Delay111/1 -> eth_cycles_per_packet/1(out_reg)
  AddSub/1 -> Delay109/1
  [eth_data_size_per_packet] -> Shift/1
  Delay109/1 -> Relational5/2, Delay111/1
  Counter25/1 -> [dsp_delay_cnt], Register1/1
  Register1/1 -> Delay153/1
  [sync_pulse] -> Counter25/1
  [acc_trig] -> Logical37/1
  [wait_for_pps] -> Counter26/1
  [acc_trig] -> Logical36/1
  Logical36/1 -> Counter26/2
  Logical37/1 -> Register1/2
  Delay143/1 -> Logical37/2
  [usec_tick] -> Counter25/2
  [rtc] -> Register2/1
  Register2/1 -> Delay154/1
  [acc_trig] -> Register2/2
  dsp_delay/1(sim_out) -> Terminator64/1
  Delay153/1 -> Delay155/1, [dsp_delay]
  Delay155/1 -> dsp_delay/1(out_reg)
  [dsp_delay] -> AddSub1/2
  Delay154/1 -> AddSub1/1
  AddSub1/1 -> [timestamp]
  Counter26/1 -> Slice28/1
  Slice28/1 -> Logical36/2, Delay143/1
  [sync_pulse] -> Counter22/1, Logical35/1
  Constant34/1 -> time_lsb/1(sim_1)
  Counter22/1 -> [rtc]
  Constant35/1 -> time_msb/1(sim_1)
  Concat8/1 -> Reinterpret8/1
  time_msb/1(in_reg) -> Concat8/1
  time_lsb/1(in_reg) -> Concat8/2
  Counter24/1 -> Relational10/1
  window_size1/1 -> Relational10/2
  Relational10/1 -> posedge18/1(in)
  posedge18/1(out) -> [usec_tick], Logical35/2, Logical38/1
  Reinterpret8/1 -> Counter22/2
  [wait_for_pps] -> Logical38/2
  Logical38/1 -> Counter24/1
  Logical35/1 -> Counter22/3
  manual_sync/1(in_reg) -> Slice2/1
  Constant40/1 -> manual_sync/1(sim_1)
  Slice2/1 -> posedge5/1(in)
  sync_next_pps/1(in_reg) -> Slice18/1
  Signal Builder1/1(Signal 1) -> sync_next_pps/1(sim_1)
  posedge16/1(out) -> Delay168/1
  Slice18/1 -> posedge16/1(in)
  Delay168/1 -> Counter18/2, [sync_next_pps]
  Logical26/1 -> [sync_pulse]
  Counter18/1 -> Slice15/1
  Delay172/1 -> Counter18/1
  Logical27/1 -> Logical26/1
  Delay117/1 -> Logical26/2
  [sync_pulse] -> Delay172/1
  posedge5/1(out) -> Delay117/1
  Logical28/1 -> Logical27/1
  Slice15/1 -> Logical27/2, [wait_for_pps]
  [timing_pps] -> Logical28/1
  [self_pps] -> Logical28/2
  Delay37/1 -> Relational/1
  Delay38/1 -> Relational/2
  Delay42/1 -> posedge1/1(in)
  Delay43/1 -> [self_pps]
  Delay45/1 -> [band_select]
  another4/1 -> stokes_snap/5(we)
  Delay83/1 -> posedge6/1(in), Delay51/1, Logical5/1
  posedge6/1(out) -> acc_snap/6(trig)
  Delay59/1 -> [vacc_1], Delay70/1, data_bus/3(in3), data_bus/1(in1)
  posedge7/1(out) -> packetiser_snap/3(trig)
  Delay46/1 -> packetiser_snap/2(we)
  packetizer/3(data_valid) -> posedge7/1(in), Delay46/1, [packetiser_dout_v]
  Delay50/1 -> packetiser_snap/1(in_word)
  Delay51/1 -> acc_snap/5(we)
  Delay57/1 -> acc_snap/4(in_rpower_odd)
  Delay58/1 -> acc_snap/3(in_rpower_even)
  Delay69/1 -> acc_snap/2(in_lpower_odd)
  Delay70/1 -> acc_snap/1(in_lpower_even)
